simulink model "r2_2f_4x_4a_4k_r366"  (R2012b)
(part 3 of 103)

      | elseif strcmp(mode, 'fields of arbitrary size')
      |     current_names = textscan(strtrim(strrep(strrep(get_param(blk, 'names'), ']', ''), '[', '')), '%s');
      |     current_names = current_names{1};
      |     numios = length(current_names);
      |     if length(current_widths) ~= numios,
      |         error('%d field names specified, but %d widths?', numios, length(current_widths));
      |     end
      | end
      | total_width = 0;
      | for ctr = 1 : length(current_widths),
      |     total_width = total_width + current_widths(ctr);
      | end
      | if total_width > 32,
      |     error('Total width must be 32 or less, set to %d.', total_width);
      | end
      mask Callback arith_types:
      | blk = gcb;
      | mode = get_param(blk, 'mode');
      | current_types = eval(get_param(blk, 'arith_types'));
      | numios = length(current_types);
      | if (strcmp(mode, 'one value') || strcmp(mode, 'fields of equal size')) && (length(current_types) > 1),
      |     error('Only one type may be specified for this mode.');
      | elseif strcmp(mode, 'fields of arbitrary size')
      |     current_names = textscan(strtrim(strrep(strrep(get_param(blk, 'names'), ']', ''), '[', '')), '%s');
      |     current_names = current_names{1};
      |     numios = length(current_names);
      |     if length(current_types) ~= numios,
      |         error('%d field names specified, but %d types?', numios, length(current_types));
      |     end
      | end
      | problem = 0;
      | for ctr = 1 : numios,
      |     t = current_types(ctr);
      |     if (t < 0) || (t > 2),
      |         problem = t;
      |         ctr = numios + 1;
      |     end
      | end
      | if problem ~= 0,
      |     error('Type cannot be %i, must be 0, 1 or 2.', problem);
      | end
      mask Callback bin_pts:
      | blk = gcb;
      | mode = get_param(blk, 'mode');
      | current_bins = eval(get_param(blk, 'bin_pts'));
      | if (strcmp(mode, 'one value') || strcmp(mode, 'fields of equal size')) && (length(current_bins) > 1),
      |     error('Only one binary pt may be specified for this mode.');
      | elseif strcmp(mode, 'fields of arbitrary size')
      |     current_names = textscan(strtrim(strrep(strrep(get_param(blk, 'names'), ']', ''), '[', '')), '%s');
      |     current_names = current_names{1};
      |     numios = length(current_names);
      |     if length(current_bins) ~= numios,
      |         error('%d field names specified, but %d binary pts?', numios, length(current_bins));
      |     end
      | end
  vacc_ld_status0 : Subsystem  Tag=xps:sw_reg  AncestorBlock=xps_library/software register  mask(swreg){mode=one value, io_dir=To Processor, io_delay=1, sample_period=1, names=reg, bitwidths=32, arith_types=0, bin_pts=0, sim_port=off, show_format=off}
      mask prompts: io_dir "I/O direction"; io_delay "I/O delay"; sample_period "Sample period"; names "Name:"; bitwidths "Bitwidth:"; arith_types "Type (ufix=0, fix=1, bool=2):"; bin_pts "Binary pt:"; sim_port "Provide sim input/output?"; show_format "Print format string?"
      mask init:
      | swreg_init(gcb)
      settings: AttributesFormatString=1output
      mask TypeOptions mode: one value | fields of equal size | fields of arbitrary size
      mask Callback mode: swreg_cb(gcb);
      mask TypeOptions io_dir: To Processor | From Processor
      mask Callback io_dir:
      | mask_enables = get_param(gcb, 'MaskEnables');
      | mask_names = get_param(gcb, 'MaskNames');
      | if strcmp(get_param(gcb, 'io_dir'), 'To Processor'),
      |     mask_enables{ismember(mask_names, 'sample_period')} = 'off';
      | else
      |     mask_enables{ismember(mask_names, 'sample_period')} = 'on';
      | end
      | set_param(gcb, 'MaskEnables', mask_enables);
      mask Callback bitwidths:
      | blk = gcb;
      | mode = get_param(blk, 'mode');
      | current_widths = eval(get_param(blk, 'bitwidths'));
      | if (strcmp(mode, 'one value') || strcmp(mode, 'fields of equal size')) && (length(current_widths) > 1),
      |     error('Only one width may be specified for this mode.');
      | elseif strcmp(mode, 'fields of arbitrary size')
      |     current_names = textscan(strtrim(strrep(strrep(get_param(blk, 'names'), ']', ''), '[', '')), '%s');
      |     current_names = current_names{1};
      |     numios = length(current_names);
      |     if length(current_widths) ~= numios,
      |         error('%d field names specified, but %d widths?', numios, length(current_widths));
      |     end
      | end
      | total_width = 0;
      | for ctr = 1 : length(current_widths),
      |     total_width = total_width + current_widths(ctr);
      | end
      | if total_width > 32,
      |     error('Total width must be 32 or less, set to %d.', total_width);
      | end
      mask Callback arith_types:
      | blk = gcb;
      | mode = get_param(blk, 'mode');
      | current_types = eval(get_param(blk, 'arith_types'));
      | numios = length(current_types);
      | if (strcmp(mode, 'one value') || strcmp(mode, 'fields of equal size')) && (length(current_types) > 1),
      |     error('Only one type may be specified for this mode.');
      | elseif strcmp(mode, 'fields of arbitrary size')
      |     current_names = textscan(strtrim(strrep(strrep(get_param(blk, 'names'), ']', ''), '[', '')), '%s');
      |     current_names = current_names{1};
      |     numios = length(current_names);
      |     if length(current_types) ~= numios,
      |         error('%d field names specified, but %d types?', numios, length(current_types));
      |     end
      | end
      | problem = 0;
      | for ctr = 1 : numios,
      |     t = current_types(ctr);
      |     if (t < 0) || (t > 2),
      |         problem = t;
      |         ctr = numios + 1;
      |     end
      | end
      | if problem ~= 0,
      |     error('Type cannot be %i, must be 0, 1 or 2.', problem);
      | end
      mask Callback bin_pts:
      | blk = gcb;
      | mode = get_param(blk, 'mode');
      | current_bins = eval(get_param(blk, 'bin_pts'));
      | if (strcmp(mode, 'one value') || strcmp(mode, 'fields of equal size')) && (length(current_bins) > 1),
      |     error('Only one binary pt may be specified for this mode.');
      | elseif strcmp(mode, 'fields of arbitrary size')
      |     current_names = textscan(strtrim(strrep(strrep(get_param(blk, 'names'), ']', ''), '[', '')), '%s');
      |     current_names = current_names{1};
      |     numios = length(current_names);
      |     if length(current_bins) ~= numios,
      |         error('%d field names specified, but %d binary pts?', numios, length(current_bins));
      |     end
      | end
  vacc_ld_status1 : Subsystem  Tag=xps:sw_reg  AncestorBlock=xps_library/software register  mask(swreg){mode=one value, io_dir=To Processor, io_delay=1, sample_period=1, names=reg, bitwidths=32, arith_types=0, bin_pts=0, sim_port=off, show_format=off}
      mask prompts: io_dir "I/O direction"; io_delay "I/O delay"; sample_period "Sample period"; names "Name:"; bitwidths "Bitwidth:"; arith_types "Type (ufix=0, fix=1, bool=2):"; bin_pts "Binary pt:"; sim_port "Provide sim input/output?"; show_format "Print format string?"
      mask init:
      | swreg_init(gcb)
      settings: AttributesFormatString=1output
      mask TypeOptions mode: one value | fields of equal size | fields of arbitrary size
      mask Callback mode: swreg_cb(gcb);
      mask TypeOptions io_dir: To Processor | From Processor
      mask Callback io_dir:
      | mask_enables = get_param(gcb, 'MaskEnables');
      | mask_names = get_param(gcb, 'MaskNames');
      | if strcmp(get_param(gcb, 'io_dir'), 'To Processor'),
      |     mask_enables{ismember(mask_names, 'sample_period')} = 'off';
      | else
      |     mask_enables{ismember(mask_names, 'sample_period')} = 'on';
      | end
      | set_param(gcb, 'MaskEnables', mask_enables);
      mask Callback bitwidths:
      | blk = gcb;
      | mode = get_param(blk, 'mode');
      | current_widths = eval(get_param(blk, 'bitwidths'));
      | if (strcmp(mode, 'one value') || strcmp(mode, 'fields of equal size')) && (length(current_widths) > 1),
      |     error('Only one width may be specified for this mode.');
      | elseif strcmp(mode, 'fields of arbitrary size')
      |     current_names = textscan(strtrim(strrep(strrep(get_param(blk, 'names'), ']', ''), '[', '')), '%s');
      |     current_names = current_names{1};
      |     numios = length(current_names);
      |     if length(current_widths) ~= numios,
      |         error('%d field names specified, but %d widths?', numios, length(current_widths));
      |     end
      | end
      | total_width = 0;
      | for ctr = 1 : length(current_widths),
      |     total_width = total_width + current_widths(ctr);
      | end
      | if total_width > 32,
      |     error('Total width must be 32 or less, set to %d.', total_width);
      | end
      mask Callback arith_types:
      | blk = gcb;
      | mode = get_param(blk, 'mode');
      | current_types = eval(get_param(blk, 'arith_types'));
      | numios = length(current_types);
      | if (strcmp(mode, 'one value') || strcmp(mode, 'fields of equal size')) && (length(current_types) > 1),
      |     error('Only one type may be specified for this mode.');
      | elseif strcmp(mode, 'fields of arbitrary size')
      |     current_names = textscan(strtrim(strrep(strrep(get_param(blk, 'names'), ']', ''), '[', '')), '%s');
      |     current_names = current_names{1};
      |     numios = length(current_names);
      |     if length(current_types) ~= numios,
      |         error('%d field names specified, but %d types?', numios, length(current_types));
      |     end
      | end
      | problem = 0;
      | for ctr = 1 : numios,
      |     t = current_types(ctr);
      |     if (t < 0) || (t > 2),
      |         problem = t;
      |         ctr = numios + 1;
      |     end
      | end
      | if problem ~= 0,
      |     error('Type cannot be %i, must be 0, 1 or 2.', problem);
      | end
      mask Callback bin_pts:
      | blk = gcb;
      | mode = get_param(blk, 'mode');
      | current_bins = eval(get_param(blk, 'bin_pts'));
      | if (strcmp(mode, 'one value') || strcmp(mode, 'fields of equal size')) && (length(current_bins) > 1),
      |     error('Only one binary pt may be specified for this mode.');
      | elseif strcmp(mode, 'fields of arbitrary size')
      |     current_names = textscan(strtrim(strrep(strrep(get_param(blk, 'names'), ']', ''), '[', '')), '%s');
      |     current_names = current_names{1};
      |     numios = length(current_names);
      |     if length(current_bins) ~= numios,
      |         error('%d field names specified, but %d binary pts?', numios, length(current_bins));
      |     end
      | end
  vacc_ld_status2 : Subsystem  Tag=xps:sw_reg  AncestorBlock=xps_library/software register  mask(swreg){mode=one value, io_dir=To Processor, io_delay=1, sample_period=1, names=reg, bitwidths=32, arith_types=0, bin_pts=0, sim_port=off, show_format=off}
      mask prompts: io_dir "I/O direction"; io_delay "I/O delay"; sample_period "Sample period"; names "Name:"; bitwidths "Bitwidth:"; arith_types "Type (ufix=0, fix=1, bool=2):"; bin_pts "Binary pt:"; sim_port "Provide sim input/output?"; show_format "Print format string?"
      mask init:
      | swreg_init(gcb)
      settings: AttributesFormatString=1output
      mask TypeOptions mode: one value | fields of equal size | fields of arbitrary size
      mask Callback mode: swreg_cb(gcb);
      mask TypeOptions io_dir: To Processor | From Processor
      mask Callback io_dir:
      | mask_enables = get_param(gcb, 'MaskEnables');
      | mask_names = get_param(gcb, 'MaskNames');
      | if strcmp(get_param(gcb, 'io_dir'), 'To Processor'),
      |     mask_enables{ismember(mask_names, 'sample_period')} = 'off';
      | else
      |     mask_enables{ismember(mask_names, 'sample_period')} = 'on';
      | end
      | set_param(gcb, 'MaskEnables', mask_enables);
      mask Callback bitwidths:
      | blk = gcb;
      | mode = get_param(blk, 'mode');
      | current_widths = eval(get_param(blk, 'bitwidths'));
      | if (strcmp(mode, 'one value') || strcmp(mode, 'fields of equal size')) && (length(current_widths) > 1),
      |     error('Only one width may be specified for this mode.');
      | elseif strcmp(mode, 'fields of arbitrary size')
      |     current_names = textscan(strtrim(strrep(strrep(get_param(blk, 'names'), ']', ''), '[', '')), '%s');
      |     current_names = current_names{1};
      |     numios = length(current_names);
      |     if length(current_widths) ~= numios,
      |         error('%d field names specified, but %d widths?', numios, length(current_widths));
      |     end
      | end
      | total_width = 0;
      | for ctr = 1 : length(current_widths),
      |     total_width = total_width + current_widths(ctr);
      | end
      | if total_width > 32,
      |     error('Total width must be 32 or less, set to %d.', total_width);
      | end
      mask Callback arith_types:
      | blk = gcb;
      | mode = get_param(blk, 'mode');
      | current_types = eval(get_param(blk, 'arith_types'));
      | numios = length(current_types);
      | if (strcmp(mode, 'one value') || strcmp(mode, 'fields of equal size')) && (length(current_types) > 1),
      |     error('Only one type may be specified for this mode.');
      | elseif strcmp(mode, 'fields of arbitrary size')
      |     current_names = textscan(strtrim(strrep(strrep(get_param(blk, 'names'), ']', ''), '[', '')), '%s');
      |     current_names = current_names{1};
      |     numios = length(current_names);
      |     if length(current_types) ~= numios,
      |         error('%d field names specified, but %d types?', numios, length(current_types));
      |     end
      | end
      | problem = 0;
      | for ctr = 1 : numios,
      |     t = current_types(ctr);
      |     if (t < 0) || (t > 2),
      |         problem = t;
      |         ctr = numios + 1;
      |     end
      | end
      | if problem ~= 0,
      |     error('Type cannot be %i, must be 0, 1 or 2.', problem);
      | end
      mask Callback bin_pts:
      | blk = gcb;
      | mode = get_param(blk, 'mode');
      | current_bins = eval(get_param(blk, 'bin_pts'));
      | if (strcmp(mode, 'one value') || strcmp(mode, 'fields of equal size')) && (length(current_bins) > 1),
      |     error('Only one binary pt may be specified for this mode.');
      | elseif strcmp(mode, 'fields of arbitrary size')
      |     current_names = textscan(strtrim(strrep(strrep(get_param(blk, 'names'), ']', ''), '[', '')), '%s');
      |     current_names = current_names{1};
      |     numios = length(current_names);
      |     if length(current_bins) ~= numios,
      |         error('%d field names specified, but %d binary pts?', numios, length(current_bins));
      |     end
      | end
  vacc_ld_status3 : Subsystem  Tag=xps:sw_reg  AncestorBlock=xps_library/software register  mask(swreg){mode=one value, io_dir=To Processor, io_delay=1, sample_period=1, names=reg, bitwidths=32, arith_types=0, bin_pts=0, sim_port=off, show_format=off}
      mask prompts: io_dir "I/O direction"; io_delay "I/O delay"; sample_period "Sample period"; names "Name:"; bitwidths "Bitwidth:"; arith_types "Type (ufix=0, fix=1, bool=2):"; bin_pts "Binary pt:"; sim_port "Provide sim input/output?"; show_format "Print format string?"
      mask init:
      | swreg_init(gcb)
      settings: AttributesFormatString=1output
      mask TypeOptions mode: one value | fields of equal size | fields of arbitrary size
      mask Callback mode: swreg_cb(gcb);
      mask TypeOptions io_dir: To Processor | From Processor
      mask Callback io_dir:
      | mask_enables = get_param(gcb, 'MaskEnables');
      | mask_names = get_param(gcb, 'MaskNames');
      | if strcmp(get_param(gcb, 'io_dir'), 'To Processor'),
      |     mask_enables{ismember(mask_names, 'sample_period')} = 'off';
      | else
      |     mask_enables{ismember(mask_names, 'sample_period')} = 'on';
      | end
      | set_param(gcb, 'MaskEnables', mask_enables);
      mask Callback bitwidths:
      | blk = gcb;
      | mode = get_param(blk, 'mode');
      | current_widths = eval(get_param(blk, 'bitwidths'));
      | if (strcmp(mode, 'one value') || strcmp(mode, 'fields of equal size')) && (length(current_widths) > 1),
      |     error('Only one width may be specified for this mode.');
      | elseif strcmp(mode, 'fields of arbitrary size')
      |     current_names = textscan(strtrim(strrep(strrep(get_param(blk, 'names'), ']', ''), '[', '')), '%s');
      |     current_names = current_names{1};
      |     numios = length(current_names);
      |     if length(current_widths) ~= numios,
      |         error('%d field names specified, but %d widths?', numios, length(current_widths));
      |     end
      | end
      | total_width = 0;
      | for ctr = 1 : length(current_widths),
      |     total_width = total_width + current_widths(ctr);
      | end
      | if total_width > 32,
      |     error('Total width must be 32 or less, set to %d.', total_width);
      | end
      mask Callback arith_types:
      | blk = gcb;
      | mode = get_param(blk, 'mode');
      | current_types = eval(get_param(blk, 'arith_types'));
      | numios = length(current_types);
      | if (strcmp(mode, 'one value') || strcmp(mode, 'fields of equal size')) && (length(current_types) > 1),
      |     error('Only one type may be specified for this mode.');
      | elseif strcmp(mode, 'fields of arbitrary size')
      |     current_names = textscan(strtrim(strrep(strrep(get_param(blk, 'names'), ']', ''), '[', '')), '%s');
      |     current_names = current_names{1};
      |     numios = length(current_names);
      |     if length(current_types) ~= numios,
      |         error('%d field names specified, but %d types?', numios, length(current_types));
      |     end
      | end
      | problem = 0;
      | for ctr = 1 : numios,
      |     t = current_types(ctr);
      |     if (t < 0) || (t > 2),
      |         problem = t;
      |         ctr = numios + 1;
      |     end
      | end
      | if problem ~= 0,
      |     error('Type cannot be %i, must be 0, 1 or 2.', problem);
      | end
      mask Callback bin_pts:
      | blk = gcb;
      | mode = get_param(blk, 'mode');
      | current_bins = eval(get_param(blk, 'bin_pts'));
      | if (strcmp(mode, 'one value') || strcmp(mode, 'fields of equal size')) && (length(current_bins) > 1),
      |     error('Only one binary pt may be specified for this mode.');
      | elseif strcmp(mode, 'fields of arbitrary size')
      |     current_names = textscan(strtrim(strrep(strrep(get_param(blk, 'names'), ']', ''), '[', '')), '%s');
      |     current_names = current_names{1};
      |     numios = length(current_names);
      |     if length(current_bins) ~= numios,
      |         error('%d field names specified, but %d binary pts?', numios, length(current_bins));
      |     end
      | end
  vacc_monitor : Subsystem
  vacc_monitor1 : Subsystem
  vacc_monitor2 : Subsystem
  vacc_monitor3 : Subsystem
  vacc_monitor4 : Subsystem
  vacc_monitor5 : Subsystem
  vacc_monitor6 : Subsystem
  vacc_monitor7 : Subsystem
  vacc_time_lsw : Subsystem  Tag=xps:sw_reg  AncestorBlock=xps_library/software register  mask(swreg){mode=one value, io_dir=From Processor, io_delay=1, sample_period=1, names=reg, bitwidths=32, arith_types=0, bin_pts=0, sim_port=on, show_format=off}
      mask prompts: io_dir "I/O direction"; io_delay "I/O delay"; sample_period "Sample period"; names "Name:"; bitwidths "Bitwidth:"; arith_types "Type (ufix=0, fix=1, bool=2):"; bin_pts "Binary pt:"; sim_port "Provide sim input/output?"; show_format "Print format string?"
      mask init:
      | swreg_init(gcb)
      settings: AttributesFormatString=1input
      mask TypeOptions mode: one value | fields of equal size | fields of arbitrary size
      mask Callback mode: swreg_cb(gcb);
      mask TypeOptions io_dir: To Processor | From Processor
      mask Callback io_dir:
      | mask_enables = get_param(gcb, 'MaskEnables');
      | mask_names = get_param(gcb, 'MaskNames');
      | if strcmp(get_param(gcb, 'io_dir'), 'To Processor'),
      |     mask_enables{ismember(mask_names, 'sample_period')} = 'off';
      | else
      |     mask_enables{ismember(mask_names, 'sample_period')} = 'on';
      | end
      | set_param(gcb, 'MaskEnables', mask_enables);
      mask Callback bitwidths:
      | blk = gcb;
      | mode = get_param(blk, 'mode');
      | current_widths = eval(get_param(blk, 'bitwidths'));
      | if (strcmp(mode, 'one value') || strcmp(mode, 'fields of equal size')) && (length(current_widths) > 1),
      |     error('Only one width may be specified for this mode.');
      | elseif strcmp(mode, 'fields of arbitrary size')
      |     current_names = textscan(strtrim(strrep(strrep(get_param(blk, 'names'), ']', ''), '[', '')), '%s');
      |     current_names = current_names{1};
      |     numios = length(current_names);
      |     if length(current_widths) ~= numios,
      |         error('%d field names specified, but %d widths?', numios, length(current_widths));
      |     end
      | end
      | total_width = 0;
      | for ctr = 1 : length(current_widths),
      |     total_width = total_width + current_widths(ctr);
      | end
      | if total_width > 32,
      |     error('Total width must be 32 or less, set to %d.', total_width);
      | end
      mask Callback arith_types:
      | blk = gcb;
      | mode = get_param(blk, 'mode');
      | current_types = eval(get_param(blk, 'arith_types'));
      | numios = length(current_types);
      | if (strcmp(mode, 'one value') || strcmp(mode, 'fields of equal size')) && (length(current_types) > 1),
      |     error('Only one type may be specified for this mode.');
      | elseif strcmp(mode, 'fields of arbitrary size')
      |     current_names = textscan(strtrim(strrep(strrep(get_param(blk, 'names'), ']', ''), '[', '')), '%s');
      |     current_names = current_names{1};
      |     numios = length(current_names);
      |     if length(current_types) ~= numios,
      |         error('%d field names specified, but %d types?', numios, length(current_types));
      |     end
      | end
      | problem = 0;
      | for ctr = 1 : numios,
      |     t = current_types(ctr);
      |     if (t < 0) || (t > 2),
      |         problem = t;
      |         ctr = numios + 1;
      |     end
      | end
      | if problem ~= 0,
      |     error('Type cannot be %i, must be 0, 1 or 2.', problem);
      | end
      mask Callback bin_pts:
      | blk = gcb;
      | mode = get_param(blk, 'mode');
      | current_bins = eval(get_param(blk, 'bin_pts'));
      | if (strcmp(mode, 'one value') || strcmp(mode, 'fields of equal size')) && (length(current_bins) > 1),
      |     error('Only one binary pt may be specified for this mode.');
      | elseif strcmp(mode, 'fields of arbitrary size')
      |     current_names = textscan(strtrim(strrep(strrep(get_param(blk, 'names'), ']', ''), '[', '')), '%s');
      |     current_names = current_names{1};
      |     numios = length(current_names);
      |     if length(current_bins) ~= numios,
      |         error('%d field names specified, but %d binary pts?', numios, length(current_bins));
      |     end
      | end
  vacc_time_msw : Subsystem  Tag=xps:sw_reg  AncestorBlock=xps_library/software register  mask(swreg){mode=fields of arbitrary size, io_dir=From Processor, io_delay=1, sample_period=1, names=[arm msw], bitwidths=[1 16], arith_types=[2 0], bin_pts=[0 0], sim_port=off, show_format=off}
      mask prompts: io_dir "I/O direction"; io_delay "I/O delay"; sample_period "Sample period"; names "Names [msb ... lsb]:"; bitwidths "Bitwidths [msb ... lsb]:"; arith_types "Types (ufix=0, fix=1, bool=2) [msb ... lsb]:"; bin_pts "Binary pts [msb ... lsb]:"; sim_port "Provide sim input/output?"; show_format "Print format string?"
      mask init:
      | swreg_init(gcb)
      settings: AttributesFormatString=2 inputs
      mask TypeOptions mode: one value | fields of equal size | fields of arbitrary size
      mask Callback mode: swreg_cb(gcb);
      mask TypeOptions io_dir: To Processor | From Processor
      mask Callback io_dir:
      | mask_enables = get_param(gcb, 'MaskEnables');
      | mask_names = get_param(gcb, 'MaskNames');
      | if strcmp(get_param(gcb, 'io_dir'), 'To Processor'),
      |     mask_enables{ismember(mask_names, 'sample_period')} = 'off';
      | else
      |     mask_enables{ismember(mask_names, 'sample_period')} = 'on';
      | end
      | set_param(gcb, 'MaskEnables', mask_enables);
      mask Callback bitwidths:
      | blk = gcb;
      | mode = get_param(blk, 'mode');
      | current_widths = eval(get_param(blk, 'bitwidths'));
      | if (strcmp(mode, 'one value') || strcmp(mode, 'fields of equal size')) && (length(current_widths) > 1),
      |     error('Only one width may be specified for this mode.');
      | elseif strcmp(mode, 'fields of arbitrary size')
      |     current_names = textscan(strtrim(strrep(strrep(get_param(blk, 'names'), ']', ''), '[', '')), '%s');
      |     current_names = current_names{1};
      |     numios = length(current_names);
      |     if length(current_widths) ~= numios,
      |         error('%d field names specified, but %d widths?', numios, length(current_widths));
      |     end
      | end
      | total_width = 0;
      | for ctr = 1 : length(current_widths),
      |     total_width = total_width + current_widths(ctr);
      | end
      | if total_width > 32,
      |     error('Total width must be 32 or less, set to %d.', total_width);
      | end
      mask Callback arith_types:
      | blk = gcb;
      | mode = get_param(blk, 'mode');
      | current_types = eval(get_param(blk, 'arith_types'));
      | numios = length(current_types);
      | if (strcmp(mode, 'one value') || strcmp(mode, 'fields of equal size')) && (length(current_types) > 1),
      |     error('Only one type may be specified for this mode.');
      | elseif strcmp(mode, 'fields of arbitrary size')
      |     current_names = textscan(strtrim(strrep(strrep(get_param(blk, 'names'), ']', ''), '[', '')), '%s');
      |     current_names = current_names{1};
      |     numios = length(current_names);
      |     if length(current_types) ~= numios,
      |         error('%d field names specified, but %d types?', numios, length(current_types));
      |     end
      | end
      | problem = 0;
      | for ctr = 1 : numios,
      |     t = current_types(ctr);
      |     if (t < 0) || (t > 2),
      |         problem = t;
      |         ctr = numios + 1;
      |     end
      | end
      | if problem ~= 0,
      |     error('Type cannot be %i, must be 0, 1 or 2.', problem);
      | end
      mask Callback bin_pts:
      | blk = gcb;
      | mode = get_param(blk, 'mode');
      | current_bins = eval(get_param(blk, 'bin_pts'));
      | if (strcmp(mode, 'one value') || strcmp(mode, 'fields of equal size')) && (length(current_bins) > 1),
      |     error('Only one binary pt may be specified for this mode.');
      | elseif strcmp(mode, 'fields of arbitrary size')
      |     current_names = textscan(strtrim(strrep(strrep(get_param(blk, 'names'), ']', ''), '[', '')), '%s');
      |     current_names = current_names{1};
      |     numios = length(current_names);
      |     if length(current_bins) ~= numios,
      |         error('%d field names specified, but %d binary pts?', numios, length(current_bins));
      |     end
      | end
  vacc_tvg0 : Subsystem  AncestorBlock=casper_library/Accumulators/vacc_tvg  mask{len=(4*(4+1))/2*8*2^(12-4)}
      mask prompts: len "Number of Vectors"
      mask init:
      | fmtstr = sprintf('Vector Length: %d', len);
      | set_param(gcb, 'AttributesFormatString', fmtstr);
      settings: AttributesFormatString=Vector Length: 20480
  vacc_tvg1 : Subsystem  AncestorBlock=casper_library/Accumulators/vacc_tvg  mask{len=(4*(4+1))/2*8*2^(12-4)}
      mask prompts: len "Number of Vectors"
      mask init:
      | fmtstr = sprintf('Vector Length: %d', len);
      | set_param(gcb, 'AttributesFormatString', fmtstr);
      settings: AttributesFormatString=Vector Length: 20480
  vacc_tvg2 : Subsystem  AncestorBlock=casper_library/Accumulators/vacc_tvg  mask{len=(4*(4+1))/2*8*2^(12-4)}
      mask prompts: len "Number of Vectors"
      mask init:
      | fmtstr = sprintf('Vector Length: %d', len);
      | set_param(gcb, 'AttributesFormatString', fmtstr);
      settings: AttributesFormatString=Vector Length: 20480
  vacc_tvg3 : Subsystem  AncestorBlock=casper_library/Accumulators/vacc_tvg  mask{len=(4*(4+1))/2*8*2^(12-4)}
      mask prompts: len "Number of Vectors"
      mask init:
      | fmtstr = sprintf('Vector Length: %d', len);
      | set_param(gcb, 'AttributesFormatString', fmtstr);
      settings: AttributesFormatString=Vector Length: 20480
  xeng0 : Subsystem  Tag=casper:xeng  AncestorBlock=casper_library_correlator/xeng  mask(xeng){n_ants=4, n_bits=8, acc_len=256, demux_factor=8, add_latency=2, mult_latency=4, bram_latency=6, use_ded_mult=1, use_bram_delay=1}
      mask prompts: n_ants "Number of antennas"; n_bits "Bit-width of samples in"; acc_len "Accumulation length"; add_latency "Adder latency"; mult_latency "Multiplier latency"; bram_latency "BRAM latency"; use_ded_mult "Implementation: Multiplier type (0=slices 1=embedded 2=bram)"; use_bram_delay "Implementation: Delay type (0=SLR, 1=BRAM)"
      mask help: CASPER X engine with added internal valid data masking functionality, descramble and integral demux. Based on Aaron Parsons' and Lynn Urry's original X engine design.
      mask init:
      | xeng_init(gcb, ...
      |     'n_ants', n_ants, ...
      |     'n_bits', n_bits, ...
      |     'acc_len', acc_len, ...
      |     'demux_factor', demux_factor, ...
      |     'add_latency', add_latency, ...
      |     'mult_latency', mult_latency, ...
      |     'bram_latency', bram_latency, ...
      |     'use_ded_mult', use_ded_mult, ...
      |     'use_bram_delay', use_bram_delay);
      settings: AttributesFormatString=n_ant=4, bits=8, mult_typ=1, bram_typ=1
      mask TypeOptions demux_factor: 1 | 2 | 4 | 8
  xeng1 : Subsystem  Tag=casper:xeng  AncestorBlock=casper_library_correlator/xeng  mask(xeng){n_ants=4, n_bits=8, acc_len=256, demux_factor=8, add_latency=2, mult_latency=4, bram_latency=6, use_ded_mult=1, use_bram_delay=1}
      mask prompts: n_ants "Number of antennas"; n_bits "Bit-width of samples in"; acc_len "Accumulation length"; add_latency "Adder latency"; mult_latency "Multiplier latency"; bram_latency "BRAM latency"; use_ded_mult "Implementation: Multiplier type (0=slices 1=embedded 2=bram)"; use_bram_delay "Implementation: Delay type (0=SLR, 1=BRAM)"
      mask help: CASPER X engine with added internal valid data masking functionality, descramble and integral demux. Based on Aaron Parsons' and Lynn Urry's original X engine design.
      mask init: same as r2_2f_4x_4a_4k_r366/xeng0
      settings: AttributesFormatString=n_ant=4, bits=8, mult_typ=1, bram_typ=1
      mask TypeOptions demux_factor: 1 | 2 | 4 | 8
  xeng2 : Subsystem  Tag=casper:xeng  AncestorBlock=casper_library_correlator/xeng  mask(xeng){n_ants=4, n_bits=8, acc_len=256, demux_factor=8, add_latency=2, mult_latency=4, bram_latency=6, use_ded_mult=1, use_bram_delay=1}
      mask prompts: n_ants "Number of antennas"; n_bits "Bit-width of samples in"; acc_len "Accumulation length"; add_latency "Adder latency"; mult_latency "Multiplier latency"; bram_latency "BRAM latency"; use_ded_mult "Implementation: Multiplier type (0=slices 1=embedded 2=bram)"; use_bram_delay "Implementation: Delay type (0=SLR, 1=BRAM)"
      mask help: CASPER X engine with added internal valid data masking functionality, descramble and integral demux. Based on Aaron Parsons' and Lynn Urry's original X engine design.
      mask init: same as r2_2f_4x_4a_4k_r366/xeng0
      settings: AttributesFormatString=n_ant=4, bits=8, mult_typ=1, bram_typ=1
      mask TypeOptions demux_factor: 1 | 2 | 4 | 8
  xeng3 : Subsystem  Tag=casper:xeng  AncestorBlock=casper_library_correlator/xeng  mask(xeng){n_ants=4, n_bits=8, acc_len=256, demux_factor=8, add_latency=2, mult_latency=4, bram_latency=6, use_ded_mult=1, use_bram_delay=1}
      mask prompts: n_ants "Number of antennas"; n_bits "Bit-width of samples in"; acc_len "Accumulation length"; add_latency "Adder latency"; mult_latency "Multiplier latency"; bram_latency "BRAM latency"; use_ded_mult "Implementation: Multiplier type (0=slices 1=embedded 2=bram)"; use_bram_delay "Implementation: Delay type (0=SLR, 1=BRAM)"
      mask help: CASPER X engine with added internal valid data masking functionality, descramble and integral demux. Based on Aaron Parsons' and Lynn Urry's original X engine design.
      mask init: same as r2_2f_4x_4a_4k_r366/xeng0
      settings: AttributesFormatString=n_ant=4, bits=8, mult_typ=1, bram_typ=1
      mask TypeOptions demux_factor: 1 | 2 | 4 | 8
  xeng_tvg0 : Subsystem  AncestorBlock=casper_library/Correlator/xeng_tvg  mask{ant_bits=2, x_int_bits=8, sync_period=16}
      mask prompts: ant_bits "Number of Antennas (2^?):"; x_int_bits "X Integration Length (2^?):"; sync_period "Sync Pulse Period (2^?):"
  xeng_tvg1 : Subsystem  AncestorBlock=casper_library/Correlator/xeng_tvg  mask{ant_bits=2, x_int_bits=8, sync_period=16}
      mask prompts: ant_bits "Number of Antennas (2^?):"; x_int_bits "X Integration Length (2^?):"; sync_period "Sync Pulse Period (2^?):"
  xeng_tvg2 : Subsystem  AncestorBlock=casper_library/Correlator/xeng_tvg  mask{ant_bits=2, x_int_bits=8, sync_period=16}
      mask prompts: ant_bits "Number of Antennas (2^?):"; x_int_bits "X Integration Length (2^?):"; sync_period "Sync Pulse Period (2^?):"
  xeng_tvg3 : Subsystem  AncestorBlock=casper_library/Correlator/xeng_tvg  mask{ant_bits=2, x_int_bits=8, sync_period=16}
      mask prompts: ant_bits "Number of Antennas (2^?):"; x_int_bits "X Integration Length (2^?):"; sync_period "Sync Pulse Period (2^?):"
  xstatus0 : Subsystem  Tag=xps:sw_reg  AncestorBlock=xps_library/software register  mask(swreg){mode=fields of equal size, io_dir=To Processor, io_delay=1, sample_period=1, names=[gbe_down rx_dest_err feng_rx_err fft_err feng_qdr_err feng_chk_err adc_over noise_diode_en vacc_err rx_bad_pkt rx_bad_frame tx_over xeng_bad_dat pack_err], bitwidths=1, arith_types=2, bin_pts=0, sim_port=off, show_format=off}
      mask prompts: io_dir "I/O direction"; io_delay "I/O delay"; sample_period "Sample period"; names "Names [msb ... lsb]:"; bitwidths "Bitwidth:"; arith_types "Type (ufix=0, fix=1, bool=2):"; bin_pts "Binary pt:"; sim_port "Provide sim input/output?"; show_format "Print format string?"
      mask init:
      | swreg_init(gcb)
      settings: AttributesFormatString=14 outputs
      mask TypeOptions mode: one value | fields of equal size | fields of arbitrary size
      mask Callback mode: swreg_cb(gcb);
      mask TypeOptions io_dir: To Processor | From Processor
      mask Callback io_dir:
      | mask_enables = get_param(gcb, 'MaskEnables');
      | mask_names = get_param(gcb, 'MaskNames');
      | if strcmp(get_param(gcb, 'io_dir'), 'To Processor'),
      |     mask_enables{ismember(mask_names, 'sample_period')} = 'off';
      | else
      |     mask_enables{ismember(mask_names, 'sample_period')} = 'on';
      | end
      | set_param(gcb, 'MaskEnables', mask_enables);
      mask Callback bitwidths:
      | blk = gcb;
      | mode = get_param(blk, 'mode');
      | current_widths = eval(get_param(blk, 'bitwidths'));
      | if (strcmp(mode, 'one value') || strcmp(mode, 'fields of equal size')) && (length(current_widths) > 1),
      |     error('Only one width may be specified for this mode.');
      | elseif strcmp(mode, 'fields of arbitrary size')
      |     current_names = textscan(strtrim(strrep(strrep(get_param(blk, 'names'), ']', ''), '[', '')), '%s');
      |     current_names = current_names{1};
      |     numios = length(current_names);
      |     if length(current_widths) ~= numios,
      |         error('%d field names specified, but %d widths?', numios, length(current_widths));
      |     end
      | end
      | total_width = 0;
      | for ctr = 1 : length(current_widths),
      |     total_width = total_width + current_widths(ctr);
      | end
      | if total_width > 32,
      |     error('Total width must be 32 or less, set to %d.', total_width);
      | end
      mask Callback arith_types:
      | blk = gcb;
      | mode = get_param(blk, 'mode');
      | current_types = eval(get_param(blk, 'arith_types'));
      | numios = length(current_types);
      | if (strcmp(mode, 'one value') || strcmp(mode, 'fields of equal size')) && (length(current_types) > 1),
      |     error('Only one type may be specified for this mode.');
      | elseif strcmp(mode, 'fields of arbitrary size')
      |     current_names = textscan(strtrim(strrep(strrep(get_param(blk, 'names'), ']', ''), '[', '')), '%s');
      |     current_names = current_names{1};
      |     numios = length(current_names);
      |     if length(current_types) ~= numios,
      |         error('%d field names specified, but %d types?', numios, length(current_types));
      |     end
      | end
      | problem = 0;
      | for ctr = 1 : numios,
      |     t = current_types(ctr);
      |     if (t < 0) || (t > 2),
      |         problem = t;
      |         ctr = numios + 1;
      |     end
      | end
      | if problem ~= 0,
      |     error('Type cannot be %i, must be 0, 1 or 2.', problem);
      | end
      mask Callback bin_pts:
      | blk = gcb;
      | mode = get_param(blk, 'mode');
      | current_bins = eval(get_param(blk, 'bin_pts'));
      | if (strcmp(mode, 'one value') || strcmp(mode, 'fields of equal size')) && (length(current_bins) > 1),
      |     error('Only one binary pt may be specified for this mode.');
      | elseif strcmp(mode, 'fields of arbitrary size')
      |     current_names = textscan(strtrim(strrep(strrep(get_param(blk, 'names'), ']', ''), '[', '')), '%s');
      |     current_names = current_names{1};
      |     numios = length(current_names);
      |     if length(current_bins) ~= numios,
      |         error('%d field names specified, but %d binary pts?', numios, length(current_bins));
      |     end
      | end
  xstatus1 : Subsystem  Tag=xps:sw_reg  AncestorBlock=xps_library/software register  mask(swreg){mode=fields of equal size, io_dir=To Processor, io_delay=1, sample_period=1, names=[gbe_down rx_dest_err feng_rx_err fft_err feng_qdr_err feng_chk_err adc_over noise_diode_en vacc_err rx_bad_pkt rx_bad_frame tx_over xeng_bad_dat pack_err], bitwidths=1, arith_types=2, bin_pts=0, sim_port=off, show_format=off}
      mask prompts: io_dir "I/O direction"; io_delay "I/O delay"; sample_period "Sample period"; names "Names [msb ... lsb]:"; bitwidths "Bitwidth:"; arith_types "Type (ufix=0, fix=1, bool=2):"; bin_pts "Binary pt:"; sim_port "Provide sim input/output?"; show_format "Print format string?"
      mask init:
      | swreg_init(gcb)
      settings: AttributesFormatString=14 outputs
      mask TypeOptions mode: one value | fields of equal size | fields of arbitrary size
      mask Callback mode: swreg_cb(gcb);
      mask TypeOptions io_dir: To Processor | From Processor
      mask Callback io_dir:
      | mask_enables = get_param(gcb, 'MaskEnables');
      | mask_names = get_param(gcb, 'MaskNames');
      | if strcmp(get_param(gcb, 'io_dir'), 'To Processor'),
      |     mask_enables{ismember(mask_names, 'sample_period')} = 'off';
      | else
      |     mask_enables{ismember(mask_names, 'sample_period')} = 'on';
      | end
      | set_param(gcb, 'MaskEnables', mask_enables);
      mask Callback bitwidths:
      | blk = gcb;
      | mode = get_param(blk, 'mode');
      | current_widths = eval(get_param(blk, 'bitwidths'));
      | if (strcmp(mode, 'one value') || strcmp(mode, 'fields of equal size')) && (length(current_widths) > 1),
      |     error('Only one width may be specified for this mode.');
      | elseif strcmp(mode, 'fields of arbitrary size')
      |     current_names = textscan(strtrim(strrep(strrep(get_param(blk, 'names'), ']', ''), '[', '')), '%s');
      |     current_names = current_names{1};
      |     numios = length(current_names);
      |     if length(current_widths) ~= numios,
      |         error('%d field names specified, but %d widths?', numios, length(current_widths));
      |     end
      | end
      | total_width = 0;
      | for ctr = 1 : length(current_widths),
      |     total_width = total_width + current_widths(ctr);
      | end
      | if total_width > 32,
      |     error('Total width must be 32 or less, set to %d.', total_width);
      | end
      mask Callback arith_types:
      | blk = gcb;
      | mode = get_param(blk, 'mode');
      | current_types = eval(get_param(blk, 'arith_types'));
      | numios = length(current_types);
      | if (strcmp(mode, 'one value') || strcmp(mode, 'fields of equal size')) && (length(current_types) > 1),
      |     error('Only one type may be specified for this mode.');
      | elseif strcmp(mode, 'fields of arbitrary size')
      |     current_names = textscan(strtrim(strrep(strrep(get_param(blk, 'names'), ']', ''), '[', '')), '%s');
      |     current_names = current_names{1};
      |     numios = length(current_names);
      |     if length(current_types) ~= numios,
      |         error('%d field names specified, but %d types?', numios, length(current_types));
      |     end
      | end
      | problem = 0;
      | for ctr = 1 : numios,
      |     t = current_types(ctr);
      |     if (t < 0) || (t > 2),
      |         problem = t;
      |         ctr = numios + 1;
      |     end
      | end
      | if problem ~= 0,
      |     error('Type cannot be %i, must be 0, 1 or 2.', problem);
      | end
      mask Callback bin_pts:
      | blk = gcb;
      | mode = get_param(blk, 'mode');
      | current_bins = eval(get_param(blk, 'bin_pts'));
      | if (strcmp(mode, 'one value') || strcmp(mode, 'fields of equal size')) && (length(current_bins) > 1),
      |     error('Only one binary pt may be specified for this mode.');
      | elseif strcmp(mode, 'fields of arbitrary size')
      |     current_names = textscan(strtrim(strrep(strrep(get_param(blk, 'names'), ']', ''), '[', '')), '%s');
      |     current_names = current_names{1};
      |     numios = length(current_names);
      |     if length(current_bins) ~= numios,
      |         error('%d field names specified, but %d binary pts?', numios, length(current_bins));
      |     end
      | end
  xstatus2 : Subsystem  Tag=xps:sw_reg  AncestorBlock=xps_library/software register  mask(swreg){mode=fields of equal size, io_dir=To Processor, io_delay=1, sample_period=1, names=[gbe_down rx_dest_err feng_rx_err fft_err feng_qdr_err feng_chk_err adc_over noise_diode_en vacc_err rx_bad_pkt rx_bad_frame tx_over xeng_bad_dat pack_err], bitwidths=1, arith_types=2, bin_pts=0, sim_port=off, show_format=off}
      mask prompts: io_dir "I/O direction"; io_delay "I/O delay"; sample_period "Sample period"; names "Names [msb ... lsb]:"; bitwidths "Bitwidth:"; arith_types "Type (ufix=0, fix=1, bool=2):"; bin_pts "Binary pt:"; sim_port "Provide sim input/output?"; show_format "Print format string?"
      mask init:
      | swreg_init(gcb)
      settings: AttributesFormatString=14 outputs
      mask TypeOptions mode: one value | fields of equal size | fields of arbitrary size
      mask Callback mode: swreg_cb(gcb);
      mask TypeOptions io_dir: To Processor | From Processor
      mask Callback io_dir:
      | mask_enables = get_param(gcb, 'MaskEnables');
      | mask_names = get_param(gcb, 'MaskNames');
      | if strcmp(get_param(gcb, 'io_dir'), 'To Processor'),
      |     mask_enables{ismember(mask_names, 'sample_period')} = 'off';
      | else
      |     mask_enables{ismember(mask_names, 'sample_period')} = 'on';
      | end
      | set_param(gcb, 'MaskEnables', mask_enables);
      mask Callback bitwidths:
      | blk = gcb;
      | mode = get_param(blk, 'mode');
      | current_widths = eval(get_param(blk, 'bitwidths'));
      | if (strcmp(mode, 'one value') || strcmp(mode, 'fields of equal size')) && (length(current_widths) > 1),
      |     error('Only one width may be specified for this mode.');
      | elseif strcmp(mode, 'fields of arbitrary size')
      |     current_names = textscan(strtrim(strrep(strrep(get_param(blk, 'names'), ']', ''), '[', '')), '%s');
      |     current_names = current_names{1};
      |     numios = length(current_names);
      |     if length(current_widths) ~= numios,
      |         error('%d field names specified, but %d widths?', numios, length(current_widths));
      |     end
      | end
      | total_width = 0;
      | for ctr = 1 : length(current_widths),
      |     total_width = total_width + current_widths(ctr);
      | end
      | if total_width > 32,
      |     error('Total width must be 32 or less, set to %d.', total_width);
      | end
      mask Callback arith_types:
      | blk = gcb;
      | mode = get_param(blk, 'mode');
      | current_types = eval(get_param(blk, 'arith_types'));
      | numios = length(current_types);
      | if (strcmp(mode, 'one value') || strcmp(mode, 'fields of equal size')) && (length(current_types) > 1),
      |     error('Only one type may be specified for this mode.');
      | elseif strcmp(mode, 'fields of arbitrary size')
      |     current_names = textscan(strtrim(strrep(strrep(get_param(blk, 'names'), ']', ''), '[', '')), '%s');
      |     current_names = current_names{1};
      |     numios = length(current_names);
      |     if length(current_types) ~= numios,
      |         error('%d field names specified, but %d types?', numios, length(current_types));
      |     end
      | end
      | problem = 0;
      | for ctr = 1 : numios,
      |     t = current_types(ctr);
      |     if (t < 0) || (t > 2),
      |         problem = t;
      |         ctr = numios + 1;
      |     end
      | end
      | if problem ~= 0,
      |     error('Type cannot be %i, must be 0, 1 or 2.', problem);
      | end
      mask Callback bin_pts:
      | blk = gcb;
      | mode = get_param(blk, 'mode');
      | current_bins = eval(get_param(blk, 'bin_pts'));
      | if (strcmp(mode, 'one value') || strcmp(mode, 'fields of equal size')) && (length(current_bins) > 1),
      |     error('Only one binary pt may be specified for this mode.');
      | elseif strcmp(mode, 'fields of arbitrary size')
      |     current_names = textscan(strtrim(strrep(strrep(get_param(blk, 'names'), ']', ''), '[', '')), '%s');
      |     current_names = current_names{1};
      |     numios = length(current_names);
      |     if length(current_bins) ~= numios,
      |         error('%d field names specified, but %d binary pts?', numios, length(current_bins));
      |     end
      | end
  xstatus3 : Subsystem  Tag=xps:sw_reg  AncestorBlock=xps_library/software register  mask(swreg){mode=fields of equal size, io_dir=To Processor, io_delay=1, sample_period=1, names=[gbe_down rx_dest_err feng_rx_err fft_err feng_qdr_err feng_chk_err adc_over noise_diode_en vacc_err rx_bad_pkt rx_bad_frame tx_over xeng_bad_dat pack_err], bitwidths=1, arith_types=2, bin_pts=0, sim_port=off, show_format=off}
      mask prompts: io_dir "I/O direction"; io_delay "I/O delay"; sample_period "Sample period"; names "Names [msb ... lsb]:"; bitwidths "Bitwidth:"; arith_types "Type (ufix=0, fix=1, bool=2):"; bin_pts "Binary pt:"; sim_port "Provide sim input/output?"; show_format "Print format string?"
      mask init:
      | swreg_init(gcb)
      settings: AttributesFormatString=14 outputs
      mask TypeOptions mode: one value | fields of equal size | fields of arbitrary size
      mask Callback mode: swreg_cb(gcb);
      mask TypeOptions io_dir: To Processor | From Processor
      mask Callback io_dir:
      | mask_enables = get_param(gcb, 'MaskEnables');
      | mask_names = get_param(gcb, 'MaskNames');
      | if strcmp(get_param(gcb, 'io_dir'), 'To Processor'),
      |     mask_enables{ismember(mask_names, 'sample_period')} = 'off';
      | else
      |     mask_enables{ismember(mask_names, 'sample_period')} = 'on';
      | end
      | set_param(gcb, 'MaskEnables', mask_enables);
      mask Callback bitwidths:
      | blk = gcb;
      | mode = get_param(blk, 'mode');
      | current_widths = eval(get_param(blk, 'bitwidths'));
      | if (strcmp(mode, 'one value') || strcmp(mode, 'fields of equal size')) && (length(current_widths) > 1),
      |     error('Only one width may be specified for this mode.');
      | elseif strcmp(mode, 'fields of arbitrary size')
      |     current_names = textscan(strtrim(strrep(strrep(get_param(blk, 'names'), ']', ''), '[', '')), '%s');
      |     current_names = current_names{1};
      |     numios = length(current_names);
      |     if length(current_widths) ~= numios,
      |         error('%d field names specified, but %d widths?', numios, length(current_widths));
      |     end
      | end
      | total_width = 0;
      | for ctr = 1 : length(current_widths),
      |     total_width = total_width + current_widths(ctr);
      | end
      | if total_width > 32,
      |     error('Total width must be 32 or less, set to %d.', total_width);
      | end
      mask Callback arith_types:
      | blk = gcb;
      | mode = get_param(blk, 'mode');
      | current_types = eval(get_param(blk, 'arith_types'));
      | numios = length(current_types);
      | if (strcmp(mode, 'one value') || strcmp(mode, 'fields of equal size')) && (length(current_types) > 1),
      |     error('Only one type may be specified for this mode.');
      | elseif strcmp(mode, 'fields of arbitrary size')
      |     current_names = textscan(strtrim(strrep(strrep(get_param(blk, 'names'), ']', ''), '[', '')), '%s');
      |     current_names = current_names{1};
      |     numios = length(current_names);
      |     if length(current_types) ~= numios,
      |         error('%d field names specified, but %d types?', numios, length(current_types));
      |     end
      | end
      | problem = 0;
      | for ctr = 1 : numios,
      |     t = current_types(ctr);
      |     if (t < 0) || (t > 2),
      |         problem = t;
      |         ctr = numios + 1;
      |     end
      | end
      | if problem ~= 0,
      |     error('Type cannot be %i, must be 0, 1 or 2.', problem);
      | end
      mask Callback bin_pts:
      | blk = gcb;
      | mode = get_param(blk, 'mode');
      | current_bins = eval(get_param(blk, 'bin_pts'));
      | if (strcmp(mode, 'one value') || strcmp(mode, 'fields of equal size')) && (length(current_bins) > 1),
      |     error('Only one binary pt may be specified for this mode.');
      | elseif strcmp(mode, 'fields of arbitrary size')
      |     current_names = textscan(strtrim(strrep(strrep(get_param(blk, 'names'), ']', ''), '[', '')), '%s');
      |     current_names = current_names{1};
      |     numios = length(current_names);
      |     if length(current_bins) ~= numios,
      |         error('%d field names specified, but %d binary pts?', numios, length(current_bins));
      |     end
      | end
  wires:
  Subsystem5/1(rx_cnt) -> Delay66/1(d)
  [cnt_rst] -> Subsystem5/1(rst)
  miss_cnt0/2(missing_cnt) -> Convert1/1
  [cnt_rst] -> miss_cnt0/1(rst)
  Subsystem5/2(err_cnt) -> Delay67/1(d)
  miss_cnt0/1(spectr_cnt) -> Convert/1
  Delay61/1(q) -> pkt_reord_cnt0/1(out_reg)
  Delay62/1(q) -> pkt_reord_err0/1(out_reg)
  Delay66/1(q) -> rx_cnt0/1(out_reg)
  Delay67/1(q) -> rx_err_cnt0/1(out_reg)
  pkt_reord_devel0/4(time_out) -> Slice38/1, Delay26/1(d)
  pkt_reord_devel0/1(sync_out) -> Delay20/1(d), [x_sync0], snap_reord0/11(trig), miss_cnt0/2(sync), snap_reord0/1(in_sync)
  master_reset_sim4/1 -> acc_len/1(sim_1)
  acc_len/1(in_reg) -> [acc_len]
  err_clear_sim2/1 -> Subsystem2/5(data_sel)
  err_clear_sim6/1 -> Subsystem2/4(valid_sel)
  err_clear_sim7/1 -> Subsystem2/3(inj_vector)
  err_clear_sim8/1 -> Subsystem2/2(inj_counter)
  Pulse Generator1/1 -> Subsystem2/1(new_acc)
  err_clear_sim9/1 -> Subsystem2/6(run)
  Subsystem2/1(Out1) -> Terminator37/1
  Delay17/1(q) -> negedge_delay/1(in)
  xeng_tvg0/1(sync_out) -> Delay56/1(d)
  xeng_tvg0/2(data_out) -> Delay73/1(d)
  xeng_tvg0/3(valid_out) -> Delay74/1(d)
  xeng0/1(sync_out) -> snap_xeng0/3(trig), vacc_tvg0/2(sync_in)
  xeng0/2(acc) -> 16b_32b/1(In1)
  xeng0/3(valid) -> vacc_tvg0/4(valid_in), snap_xeng0/2(we)
  [xeng_tvg_sel] -> xeng_tvg0/1(tvg_sel)
  [vacc_tvg_sel] -> vacc_tvg0/1(tvg_sel)
  Delay151/1(q) -> Delay83/1(d)
  Delay20/1(q) -> xeng_tvg0/2(sync)
  Delay21/1(q) -> xeng_tvg0/3(data_in)
  Delay22/1(q) -> xeng_tvg0/4(valid_in)
  Delay26/1(q) -> Delay151/1(d)
  Delay118/1(q) -> negedge_delay1/1(in)
  16b_32b/1(Out1) -> snap_xeng0/1(din), vacc_tvg0/3(data_in)
  Delay130/1(q) -> last_missing_ant0/1(out_reg)
  miss_cnt0/3(last_missed_ant) -> Convert2/1
  [gbe_rxvld0] -> Delay6/1(d)
  [gbe_rxdata0] -> Delay2/1(d)
  [gbe_rxeof0] -> Delay7/1(d)
  Delay2/1(q) -> spead_unpack0/1(pkt_data)
  Delay6/1(q) -> spead_unpack0/2(pkt_valid)
  Delay7/1(q) -> spead_unpack0/3(pkt_eof)
  vacc_tvg0/1(sync_out) -> fake_vacc0/5(sync_in)
  vacc_tvg0/2(data_out) -> fake_vacc0/6(data_in)
  vacc_tvg0/3(valid_out) -> fake_vacc0/7(we)
  [acc_len] -> fake_vacc0/4(acc_len)
  xeng0/4(mcnt_out) -> delay5/1
  vacc_monitor/2(spec_cnt) -> vacc_cnt0/1(out_reg)
  vacc_monitor/1(error_cnt) -> vacc_err_cnt0/1(out_reg)
  fake_vacc0/1(new_acc) -> [new_acc0]
  [cnt_rst] -> vacc_monitor/1(cnt_rst)
  fake_vacc0/7(timestamp) -> delay7/1
  Delay80/1(q) -> Subsystem5/2(we)
  Delay81/1(q) -> Subsystem5/3(eof)
  Delay82/1(q) -> Subsystem5/4(flag)
  Delay56/1(q) -> xeng0/1(sync_in)
  Delay73/1(q) -> xeng0/2(ant)
  Delay74/1(q) -> xeng0/3(window_valid)
  Delay83/1(q) -> xeng0/4(mcnt_in)
  [gbe_out_rst] -> delay8/1
  [gbe_txd0] -> delay9/1
  [gbe_txvld0] -> delay10/1
  [gbe_txip] -> delay11/1
  [gbe_txport] -> delay12/1
  [gbe_txeof0] -> delay13/1
  gbe0/1(led_up) -> [gbe_up0]
  gbe0/2(led_rx) -> Terminator7/1
  gbe0/3(led_tx) -> Terminator13/1
  gbe0/4(tx_afull) -> Terminator14/1
  gbe0/5(tx_overflow) -> [gbe_tx_over0]
  gbe0/12(rx_overrun) -> Terminator36/1
  gbe0/11(rx_bad_frame) -> [gbe_rx_bad0]
  gbe0/6(rx_data) -> [gbe_rxdata0]
  gbe0/7(rx_valid) -> [gbe_rxvld0]
  gbe0/8(rx_source_ip) -> Terminator15/1
  gbe0/9(rx_source_port) -> Terminator35/1
  gbe0/10(rx_end_of_frame) -> [gbe_rxeof0]
  [vacc_ld_arm] -> fake_vacc0/2(arm)
  [vacc_ld_time] -> fake_vacc0/3(load_time)
  [vacc_rst] -> fake_vacc0/1(rst)
  delay5/1 -> fake_vacc0/8(pcnt_in)
  fake_vacc0/10(error_out) -> [vacc_err0]
  [new_acc0] -> vacc_monitor/2(new_acc)
  [vacc_err0] -> vacc_monitor/3(error)
  pkt_reord_devel0/2(data_out) -> snap_reord0/2(in_data), Delay21/1(d)
  Delay27/1(q) -> negedge_delay2/1(in)
  Delay96/1(q) -> negedge_delay3/1(in)
  Delay97/1(q) -> negedge_delay4/1(in)
  miss_cnt0/4(not_rcvd) -> [xeng_rx_err0]
  fake_vacc0/2(data_out) -> delay4/1
  fake_vacc0/4(valid_out) -> delay2/1
  fake_vacc0/6(rb_done) -> delay6/1
  [vacc_ld_stat0] -> vacc_ld_status0/1(out_reg)
  fake_vacc0/8(ld_status) -> [vacc_ld_stat0]
  [id0] -> pack_out0/6(xeng_id)
  [vacc_err0] -> snap_vacc0/4(stop)
  pack_out0/3(eof) -> Delay15/1(d)
  [cnt_rst] -> vacc_monitor2/1(cnt_rst)
  vacc_monitor2/1(pkt_cnt) -> pack_out_cnt0/1(out_reg)
  vacc_monitor2/2(error_cnt) -> pack_out_err0/1(out_reg)
  pack_out0/5(fetch) -> fake_vacc0/9(re)
  delay4/1 -> snap_vacc0/1(din), pack_out0/1(data_in)
  delay2/1 -> snap_vacc0/2(we), pack_out0/2(valid_in)
  delay6/1 -> pack_out0/4(rb_done), snap_vacc0/3(trig)
  delay7/1 -> pack_out0/5(timestamp)
  pack_out0/1(data_out) -> Delay23/1(d)
  pack_out0/2(valid_out) -> Logical/2
  pack_out0/4(err) -> Delay34/1(d)
  Delay34/1(q) -> [pack_err0], vacc_monitor2/3(error)
  delay8/1 -> gbe0/1(rst)
  delay9/1 -> gbe0/2(tx_data)
  delay10/1 -> gbe0/3(tx_valid)
  delay11/1 -> gbe0/4(tx_dest_ip)
  delay12/1 -> gbe0/5(tx_dest_port)
  delay13/1 -> gbe0/6(tx_end_of_frame)
  Constant2/1 -> gbe0/7(rx_ack)
  Constant8/1 -> gbe0/8(rx_overrun_ack)
  Delay46/1 -> pack_out0/3(pkt_rdy)
  negedge_delay3/1(out) -> front_panel/6(led2_red)
  negedge_delay4/1(out) -> front_panel/7(led3_red)
  [flasher_en] -> front_panel/1(flasher_en)
  [new_acc0] -> front_panel/2(sync)
  [x_sync0] -> front_panel/3(step)
  negedge_delay2/1(out) -> front_panel/4(led0_red)
  negedge_delay/1(out) -> front_panel/10(led6_green)
  negedge_delay1/1(out) -> front_panel/9(led5_green)
  Delay16/1 -> [gbe_txvld0]
  Delay23/1(q) -> rate_ctrl0/1(din0)
  rate_ctrl0/2(valid) -> Delay16/1
  Constant22/1 -> [beng_data_id]
  rate_ctrl0/1(dout) -> Delay114/1
  Delay114/1 -> [gbe_txd0]
  gbe_out_port/1(in_reg) -> Delay9/1(d)
  gbe_out_ip/1(in_reg) -> Delay10/1(d)
  Delay9/1(q) -> [gbe_txport]
  Delay10/1(q) -> [gbe_txip]
  [gbe_out_en] -> Logical/1
  Constant24/1 -> [beng_time_id]
  Logical/1 -> rate_ctrl0/2(valid0)
  Delay15/1(q) -> vacc_monitor2/2(eof), rate_ctrl0/3(eof0)
  fake_vacc0/5(pkt_rdy) -> rate_ctrl0/4(data_rdy0)
  spead_unpack0/1(pkt_start) -> Terminator28/1
  pre_process0/9(dest_err) -> Logical1/2, [rx_dest_err0], snap_unpack0/9(in_dest_err)
  pre_process0/1(data_out) -> pkt_reord_devel0/1(din), snap_unpack0/1(in_data)
  pre_process0/2(valid) -> snap_unpack0/15(we), pkt_reord_devel0/2(valid_in), snap_unpack0/2(in_valid)
  pre_process0/3(eof_out) -> snap_unpack0/16(trig), pkt_reord_devel0/3(eof), snap_unpack0/3(in_eof)
  pre_process0/4(timestamp) -> pkt_reord_devel0/4(time), Slice29/1
  pre_process0/5(feng_id) -> pkt_reord_devel0/5(ant), Slice30/1
  pre_process0/6(freq_out) -> Slice31/1, pkt_reord_devel0/6(freq)
  pre_process0/8(spead_err_out) -> Logical1/1, [spead_err0], snap_unpack0/8(in_spead_err)
  pre_process0/7(adc_over) -> [adc_err0], snap_unpack0/7(in_adc_over)
  pre_process0/10(fft_err) -> snap_unpack0/10(in_fft_err), [fft_err0]
  pre_process0/11(feng_rx_err) -> snap_unpack0/11(in_feng_rx_err), Logical1/3, [feng_rx_err0]
  pre_process0/12(nd_en) -> snap_unpack0/12(in_nd_en), [noise_diode_en0]
  pkt_reord_devel0/7(err) -> Terminator2/1
  pre_process0/13(chksum_err) -> snap_unpack0/13(in_chksum_err), Logical1/4, [feng_chk_err0]
  pre_process0/14(qdr_err) -> snap_unpack0/14(in_feng_qdr_err), [feng_qdr_err0]
  [id0] -> pre_process0/9(board_id)
  Constant3/1 -> Delay72/1(d)
  Delay72/1(q) -> Subsystem1/1(In1)
  Subsystem1/1(Out1) -> [id0]
  Subsystem1/2(Out2) -> [id1]
  Subsystem1/3(Out3) -> [id2]
  Subsystem1/4(Out4) -> [id3]
  [id0] -> pkt_reord_devel0/8(board_id)
  pkt_reord_devel0/3(valid_out) -> miss_cnt0/3(valid), snap_reord0/3(in_valid), snap_reord0/10(we), Logical6/2, Delay22/1(d)
  pkt_reord_devel0/5(freq_out) -> Convert12/1
  Slice12/1 -> snap_reord0/7(in_feng_err)
  Slice16/1 -> snap_reord0/9(in_nd_on)
  Slice15/1 -> snap_reord0/8(in_adc_over)
  pkt_reord_devel0/6(flag_out) -> Slice11/1, Slice12/1, Slice15/1, Slice16/1
  Slice11/1 -> miss_cnt0/4(not rcvd), snap_reord0/6(in_xeng_err), Logical6/1
  Logical6/1 -> snap_reord0/12(stop)
  miss_cnt1/2(missing_cnt) -> Convert4/1
  [cnt_rst] -> miss_cnt1/1(rst)
  miss_cnt1/1(spectr_cnt) -> Convert3/1
  pkt_reord_devel1/4(time_out) -> Slice21/1, Delay30/1(d)
  pkt_reord_devel1/1(sync_out) -> snap_reord1/11(trig), snap_reord1/1(in_sync), miss_cnt1/2(sync), Delay5/1(d)
  xeng_tvg1/1(sync_out) -> Delay32/1(d)
  xeng_tvg1/2(data_out) -> Delay36/1(d)
  xeng_tvg1/3(valid_out) -> Delay37/1(d)
  xeng1/1(sync_out) -> vacc_tvg1/2(sync_in)
  xeng1/2(acc) -> 16b_32b1/1(In1)
  xeng1/3(valid) -> vacc_tvg1/4(valid_in)
  [xeng_tvg_sel] -> xeng_tvg1/1(tvg_sel)
  [vacc_tvg_sel] -> vacc_tvg1/1(tvg_sel)
  Delay4/1(q) -> Delay38/1(d)
  Delay5/1(q) -> xeng_tvg1/2(sync)
  Delay11/1(q) -> xeng_tvg1/3(data_in)
  Delay14/1(q) -> xeng_tvg1/4(valid_in)
  Delay30/1(q) -> Delay4/1(d)
  16b_32b1/1(Out1) -> vacc_tvg1/3(data_in)
  miss_cnt1/3(last_missed_ant) -> Convert5/1
  vacc_tvg1/1(sync_out) -> fake_vacc1/5(sync_in)
  vacc_tvg1/2(data_out) -> fake_vacc1/6(data_in)
  vacc_tvg1/3(valid_out) -> fake_vacc1/7(we)
  [acc_len] -> fake_vacc1/4(acc_len)
  xeng1/4(mcnt_out) -> delay16/1
  vacc_monitor1/2(spec_cnt) -> vacc_cnt1/1(out_reg)
  vacc_monitor1/1(error_cnt) -> vacc_err_cnt1/1(out_reg)
  fake_vacc1/1(new_acc) -> vacc_monitor1/2(new_acc), [new_acc1]
  [cnt_rst] -> vacc_monitor1/1(cnt_rst)
  fake_vacc1/7(timestamp) -> delay18/1
  Delay32/1(q) -> xeng1/1(sync_in)
  Delay36/1(q) -> xeng1/2(ant)
  Delay37/1(q) -> xeng1/3(window_valid)
  Delay38/1(q) -> xeng1/4(mcnt_in)
  [vacc_ld_arm] -> fake_vacc1/2(arm)
  [vacc_ld_time] -> fake_vacc1/3(load_time)
  [vacc_rst] -> fake_vacc1/1(rst)
  delay16/1 -> fake_vacc1/8(pcnt_in)
  pkt_reord_devel1/2(data_out) -> snap_reord1/2(in_data), Delay11/1(d)
  miss_cnt1/4(not_rcvd) -> [xeng_rx_err1]
  fake_vacc1/2(data_out) -> delay3/1
  fake_vacc1/4(valid_out) -> delay1/1
  fake_vacc1/6(rb_done) -> delay17/1
  fake_vacc1/5(pkt_rdy) -> rate_ctrl1/4(data_rdy0)
  fake_vacc1/8(ld_status) -> vacc_ld_status1/1(out_reg)
  [id1] -> pack_out1/6(xeng_id)
  fake_vacc1/10(error_out) -> snap_vacc1/4(stop), vacc_monitor1/3(error), [vacc_err1]
  pack_out1/3(eof) -> Delay3/1(d)
  [cnt_rst] -> vacc_monitor3/1(cnt_rst)
  vacc_monitor3/1(pkt_cnt) -> pack_out_cnt1/1(out_reg)
  vacc_monitor3/2(error_cnt) -> pack_out_err1/1(out_reg)
  pack_out1/5(fetch) -> fake_vacc1/9(re)
  delay3/1 -> pack_out1/1(data_in), snap_vacc1/1(din)
  delay1/1 -> pack_out1/2(valid_in), snap_vacc1/2(we)
  delay17/1 -> pack_out1/4(rb_done), snap_vacc1/3(trig)
  delay18/1 -> pack_out1/5(timestamp)
  pack_out1/1(data_out) -> Delay28/1(d)
  pack_out1/2(valid_out) -> Logical7/2
  Delay28/1(q) -> rate_ctrl1/1(din0)
  Logical7/1 -> rate_ctrl1/2(valid0)
  pack_out1/4(err) -> Delay31/1(d)
  Delay3/1(q) -> vacc_monitor3/2(eof), rate_ctrl1/3(eof0)
  Delay31/1(q) -> [pack_err1], vacc_monitor3/3(error)
  Delay42/1 -> pack_out1/3(pkt_rdy)
  [gbe_out_en] -> Logical7/1
  pkt_reord_devel1/7(err) -> Terminator20/1
  [id1] -> pkt_reord_devel1/8(board_id)
  [flags1] -> pkt_reord_devel1/7(flag)
  pkt_reord_devel1/3(valid_out) -> snap_reord1/10(we), snap_reord1/3(in_valid), miss_cnt1/3(valid), Logical8/2, Delay14/1(d)
  pkt_reord_devel1/5(freq_out) -> Convert13/1
  Slice18/1 -> snap_reord1/7(in_feng_err)
  Slice20/1 -> snap_reord1/9(in_nd_on)
  Slice19/1 -> snap_reord1/8(in_adc_over)
  pkt_reord_devel1/6(flag_out) -> Slice20/1, Slice19/1, Slice18/1, Slice17/1
  Slice17/1 -> snap_reord1/6(in_xeng_err), miss_cnt1/4(not rcvd), Logical8/1
  Logical8/1 -> snap_reord1/12(stop)
  Constant6/1 -> vacc_time_lsw/1(sim_1)
  vacc_time_msw/2(in_msw) -> Concat12/1
  vacc_time_lsw/1(in_reg) -> Concat12/2
  vacc_time_msw/1(in_arm) -> [vacc_ld_arm]
  Concat12/1 -> [vacc_ld_time]
  rate_ctrl0/3(eof) -> Delay45/1
  rate_ctrl0/4(pkt_send0) -> Delay46/1
  Delay45/1 -> [gbe_txeof0]
  Delay40/1 -> [gbe_txvld1]
  rate_ctrl1/2(valid) -> Delay40/1
  rate_ctrl1/1(dout) -> Delay39/1
  Delay39/1 -> [gbe_txd1]
  rate_ctrl1/3(eof) -> Delay41/1
  rate_ctrl1/4(pkt_send0) -> Delay42/1
  Delay41/1 -> [gbe_txeof1]
  Subsystem8/1(rx_cnt) -> Delay68/1(d)
  [cnt_rst] -> Subsystem8/1(rst)
  spead_unpack0/3(valid64) -> pre_process0/2(valid_in), Delay85/1(d), pre_process1/2(valid_in), Delay80/1(d)
  spead_unpack0/6(hdr1_0x1600) -> pre_process1/5(hdr1), pre_process0/5(hdr1)
  spead_unpack0/2(data64) -> pre_process1/1(data_in), pre_process0/1(data_in)
  spead_unpack0/4(eof64) -> pre_process0/3(eof_in), Delay90/1(d), pre_process1/3(eof_in), Delay81/1(d)
  spead_unpack0/7(hdr2_0x4101) -> pre_process1/6(hdr2), pre_process0/6(hdr2)
  Subsystem8/2(err_cnt) -> Delay69/1(d)
  spead_unpack0/8(hdr3_0x4102) -> pre_process1/7(hdr3), pre_process0/7(hdr3)
  spead_unpack0/5(error) -> pre_process0/4(spead_err), Delay91/1(d), pre_process1/4(spead_err), Delay82/1(d)
  Delay85/1(q) -> Subsystem8/2(we)
  Delay90/1(q) -> Subsystem8/3(eof)
  Delay91/1(q) -> Subsystem8/4(flag)
  spead_unpack1/1(pkt_start) -> Terminator34/1
  spead_unpack0/9(hdr4_0x4103) -> pre_process1/8(hdr4), pre_process0/8(hdr4)
  pre_process1/9(dest_err) -> [rx_dest_err1]
  pre_process1/1(data_out) -> pkt_reord_devel1/1(din)
  pre_process1/2(valid) -> pkt_reord_devel1/2(valid_in)
  pre_process1/3(eof_out) -> pkt_reord_devel1/3(eof)
  pre_process1/4(timestamp) -> pkt_reord_devel1/4(time)
  pre_process1/5(feng_id) -> pkt_reord_devel1/5(ant)
  pre_process1/6(freq_out) -> pkt_reord_devel1/6(freq)
  pre_process1/8(spead_err_out) -> [spead_err1]
  pre_process1/7(adc_over) -> [adc_err1]
  pre_process1/10(fft_err) -> [fft_err1]
  pre_process1/11(feng_rx_err) -> [feng_rx_err1]
  pre_process1/12(nd_en) -> [noise_diode_en1]
  pre_process1/13(chksum_err) -> [feng_chk_err1]
  pre_process1/14(qdr_err) -> [feng_qdr_err1]
  [id1] -> pre_process1/9(board_id)
  [gbe_out_rst] -> delay21/1
  [gbe_txd1] -> delay22/1
  [gbe_txip] -> delay15/1
  [gbe_txport] -> delay19/1
  delay21/1 -> gbe1/1(rst)
  delay22/1 -> gbe1/2(tx_data)
  delay14/1 -> gbe1/3(tx_valid)
  delay15/1 -> gbe1/4(tx_dest_ip)
  delay19/1 -> gbe1/5(tx_dest_port)
  delay20/1 -> gbe1/6(tx_end_of_frame)
  Constant9/1 -> gbe1/7(rx_ack)
  Constant13/1 -> gbe1/8(rx_overrun_ack)
  gbe1/11(rx_bad_frame) -> [gbe_rx_bad1]
  gbe1/5(tx_overflow) -> [gbe_tx_over1]
  [gbe_txeof1] -> delay20/1
  [gbe_txvld1] -> delay14/1
  miss_cnt2/2(missing_cnt) -> Convert7/1
  [cnt_rst] -> miss_cnt2/1(rst)
  miss_cnt2/1(spectr_cnt) -> Convert6/1
  pkt_reord_devel3/4(time_out) -> Slice27/1, Delay111/1(d)
  pkt_reord_devel3/1(sync_out) -> Delay133/1(d), snap_reord2/11(trig), snap_reord2/1(in_sync), miss_cnt2/2(sync)
  xeng_tvg2/1(sync_out) -> Delay113/1(d)
  xeng_tvg2/2(data_out) -> Delay119/1(d)
  xeng_tvg2/3(valid_out) -> Delay120/1(d)
  xeng2/1(sync_out) -> vacc_tvg2/2(sync_in)
  xeng2/2(acc) -> 16b_32b2/1(In1)
  xeng2/3(valid) -> vacc_tvg2/4(valid_in)
  [xeng_tvg_sel] -> xeng_tvg2/1(tvg_sel)
  [vacc_tvg_sel] -> vacc_tvg2/1(tvg_sel)
  Delay124/1(q) -> Delay121/1(d)
  Delay133/1(q) -> xeng_tvg2/2(sync)
  Delay107/1(q) -> xeng_tvg2/3(data_in)
  Delay108/1(q) -> xeng_tvg2/4(valid_in)
  Delay111/1(q) -> Delay124/1(d)
  16b_32b2/1(Out1) -> vacc_tvg2/3(data_in)
  miss_cnt2/3(last_missed_ant) -> Convert8/1
  vacc_tvg2/1(sync_out) -> fake_vacc2/5(sync_in)
  vacc_tvg2/2(data_out) -> fake_vacc2/6(data_in)
  vacc_tvg2/3(valid_out) -> fake_vacc2/7(we)
  [acc_len] -> fake_vacc2/4(acc_len)
  xeng2/4(mcnt_out) -> delay26/1
  vacc_monitor4/2(spec_cnt) -> vacc_cnt2/1(out_reg)
  vacc_monitor4/1(error_cnt) -> vacc_err_cnt2/1(out_reg)
  fake_vacc2/1(new_acc) -> [new_acc2], vacc_monitor4/2(new_acc)
  [cnt_rst] -> vacc_monitor4/1(cnt_rst)
  fake_vacc2/7(timestamp) -> delay28/1
  Delay113/1(q) -> xeng2/1(sync_in)
  Delay119/1(q) -> xeng2/2(ant)
  Delay120/1(q) -> xeng2/3(window_valid)
  Delay121/1(q) -> xeng2/4(mcnt_in)
  [vacc_ld_arm] -> fake_vacc2/2(arm)
  [vacc_ld_time] -> fake_vacc2/3(load_time)
  [vacc_rst] -> fake_vacc2/1(rst)
  delay26/1 -> fake_vacc2/8(pcnt_in)
  pkt_reord_devel3/2(data_out) -> snap_reord2/2(in_data), Delay107/1(d)
  miss_cnt2/4(not_rcvd) -> [xeng_rx_err2]
  fake_vacc2/2(data_out) -> delay33/1
  fake_vacc2/4(valid_out) -> delay23/1
  fake_vacc2/6(rb_done) -> delay27/1
  fake_vacc2/5(pkt_rdy) -> rate_ctrl2/4(data_rdy0)
  fake_vacc2/8(ld_status) -> vacc_ld_status2/1(out_reg)
  [id2] -> pack_out2/6(xeng_id)
  fake_vacc2/10(error_out) -> [vacc_err2], vacc_monitor4/3(error), snap_vacc2/4(stop)
  pack_out2/3(eof) -> Delay110/1(d)
  [cnt_rst] -> vacc_monitor5/1(cnt_rst)
  vacc_monitor5/1(pkt_cnt) -> pack_out_cnt2/1(out_reg)
  vacc_monitor5/2(error_cnt) -> pack_out_err2/1(out_reg)
  pack_out2/5(fetch) -> fake_vacc2/9(re)
  delay33/1 -> snap_vacc2/1(din), pack_out2/1(data_in)
  delay23/1 -> snap_vacc2/2(we), pack_out2/2(valid_in)
  delay27/1 -> snap_vacc2/3(trig), pack_out2/4(rb_done)
  delay28/1 -> pack_out2/5(timestamp)
  pack_out2/1(data_out) -> Delay109/1(d)
  pack_out2/2(valid_out) -> Logical12/2
  Delay109/1(q) -> rate_ctrl2/1(din0)
  Logical12/1 -> rate_ctrl2/2(valid0)
  pack_out2/4(err) -> Delay112/1(d)
  Delay110/1(q) -> rate_ctrl2/3(eof0), vacc_monitor5/2(eof)
  Delay112/1(q) -> [pack_err2], vacc_monitor5/3(error)
  Delay127/1 -> pack_out2/3(pkt_rdy)
  [gbe_out_en] -> Logical12/1
  pkt_reord_devel3/7(err) -> Terminator40/1
  [id2] -> pkt_reord_devel3/8(board_id)
  [flags2] -> pkt_reord_devel3/7(flag)
  pkt_reord_devel3/3(valid_out) -> Delay108/1(d), Logical13/2, snap_reord2/10(we), miss_cnt2/3(valid), snap_reord2/3(in_valid)
  pkt_reord_devel3/5(freq_out) -> Convert14/1
  Slice24/1 -> snap_reord2/7(in_feng_err)
  Slice26/1 -> snap_reord2/9(in_nd_on)
  Slice25/1 -> snap_reord2/8(in_adc_over)
  pkt_reord_devel3/6(flag_out) -> Slice26/1, Slice25/1, Slice23/1, Slice24/1
  Slice23/1 -> Logical13/1, snap_reord2/6(in_xeng_err), miss_cnt2/4(not rcvd)
  Logical13/1 -> snap_reord2/12(stop)
  Delay125/1 -> [gbe_txvld2]
  rate_ctrl2/2(valid) -> Delay125/1
  rate_ctrl2/1(dout) -> Delay123/1
  Delay123/1 -> [gbe_txd2]
  rate_ctrl2/3(eof) -> Delay126/1
  rate_ctrl2/4(pkt_send0) -> Delay127/1
  Delay126/1 -> [gbe_txeof2]
  Subsystem11/1(rx_cnt) -> Delay149/1(d)
  [cnt_rst] -> Subsystem11/1(rst)
  Subsystem11/2(err_cnt) -> Delay150/1(d)
  Delay149/1(q) -> rx_cnt2/1(out_reg)
  Delay150/1(q) -> rx_err_cnt2/1(out_reg)
  Delay155/1(q) -> Subsystem11/2(we)
  Delay156/1(q) -> Subsystem11/3(eof)
  Delay157/1(q) -> Subsystem11/4(flag)
  pre_process2/9(dest_err) -> [rx_dest_err2]
  pre_process2/1(data_out) -> pkt_reord_devel3/1(din)
  pre_process2/2(valid) -> pkt_reord_devel3/2(valid_in)
  pre_process2/3(eof_out) -> pkt_reord_devel3/3(eof)
  pre_process2/4(timestamp) -> pkt_reord_devel3/4(time)
  pre_process2/5(feng_id) -> pkt_reord_devel3/5(ant)
  pre_process2/6(freq_out) -> pkt_reord_devel3/6(freq)
  pre_process2/8(spead_err_out) -> [spead_err2]
  pre_process2/7(adc_over) -> [adc_err2]
  pre_process2/10(fft_err) -> [fft_err2]
  pre_process2/11(feng_rx_err) -> [feng_rx_err2]
  pre_process2/12(nd_en) -> [noise_diode_en2]
  pre_process2/13(chksum_err) -> [feng_chk_err2]
  pre_process2/14(qdr_err) -> [feng_qdr_err2]
  [id2] -> pre_process2/9(board_id)
  miss_cnt3/2(missing_cnt) -> Convert10/1
  [cnt_rst] -> miss_cnt3/1(rst)
  miss_cnt3/1(spectr_cnt) -> Convert9/1
  pkt_reord_devel4/4(time_out) -> Slice36/1, Delay171/1(d)
  pkt_reord_devel4/1(sync_out) -> Delay188/1(d), snap_reord3/11(trig), snap_reord3/1(in_sync), miss_cnt3/2(sync)
  xeng_tvg3/1(sync_out) -> Delay173/1(d)
  xeng_tvg3/2(data_out) -> Delay176/1(d)
  xeng_tvg3/3(valid_out) -> Delay177/1(d)
  xeng3/1(sync_out) -> vacc_tvg3/2(sync_in)
  xeng3/2(acc) -> 16b_32b3/1(In1)
  xeng3/3(valid) -> vacc_tvg3/4(valid_in)
  [xeng_tvg_sel] -> xeng_tvg3/1(tvg_sel)
  [vacc_tvg_sel] -> vacc_tvg3/1(tvg_sel)
  Delay180/1(q) -> Delay178/1(d)
  Delay188/1(q) -> xeng_tvg3/2(sync)
  Delay167/1(q) -> xeng_tvg3/3(data_in)
  Delay168/1(q) -> xeng_tvg3/4(valid_in)
  Delay171/1(q) -> Delay180/1(d)
  16b_32b3/1(Out1) -> vacc_tvg3/3(data_in)
  miss_cnt3/3(last_missed_ant) -> Convert11/1
  vacc_tvg3/1(sync_out) -> fake_vacc3/5(sync_in)
  vacc_tvg3/2(data_out) -> fake_vacc3/6(data_in)
  vacc_tvg3/3(valid_out) -> fake_vacc3/7(we)
  [acc_len] -> fake_vacc3/4(acc_len)
  xeng3/4(mcnt_out) -> delay37/1
  vacc_monitor6/2(spec_cnt) -> vacc_cnt3/1(out_reg)
  vacc_monitor6/1(error_cnt) -> vacc_err_cnt3/1(out_reg)
  fake_vacc3/1(new_acc) -> vacc_monitor6/2(new_acc), [new_acc3]
  [cnt_rst] -> vacc_monitor6/1(cnt_rst)
  fake_vacc3/7(timestamp) -> delay39/1
  Delay173/1(q) -> xeng3/1(sync_in)
  Delay176/1(q) -> xeng3/2(ant)
  Delay177/1(q) -> xeng3/3(window_valid)
  Delay178/1(q) -> xeng3/4(mcnt_in)
  [vacc_ld_arm] -> fake_vacc3/2(arm)
  [vacc_ld_time] -> fake_vacc3/3(load_time)
  [vacc_rst] -> fake_vacc3/1(rst)
  delay37/1 -> fake_vacc3/8(pcnt_in)
  pkt_reord_devel4/2(data_out) -> snap_reord3/2(in_data), Delay167/1(d)
  miss_cnt3/4(not_rcvd) -> [xeng_rx_err3]
  fake_vacc3/2(data_out) -> delay44/1
  fake_vacc3/4(valid_out) -> delay34/1
  fake_vacc3/6(rb_done) -> delay38/1
  fake_vacc3/5(pkt_rdy) -> rate_ctrl3/4(data_rdy0)
  fake_vacc3/8(ld_status) -> vacc_ld_status3/1(out_reg)
  [id3] -> pack_out3/6(xeng_id)
  fake_vacc3/10(error_out) -> snap_vacc3/4(stop), vacc_monitor6/3(error), [vacc_err3]
  pack_out3/3(eof) -> Delay170/1(d)
  [cnt_rst] -> vacc_monitor7/1(cnt_rst)
  vacc_monitor7/1(pkt_cnt) -> pack_out_cnt3/1(out_reg)
  vacc_monitor7/2(error_cnt) -> pack_out_err3/1(out_reg)
  pack_out3/5(fetch) -> fake_vacc3/9(re)
  delay44/1 -> pack_out3/1(data_in), snap_vacc3/1(din)
  delay34/1 -> pack_out3/2(valid_in), snap_vacc3/2(we)
  delay38/1 -> pack_out3/4(rb_done), snap_vacc3/3(trig)
  delay39/1 -> pack_out3/5(timestamp)
  pack_out3/1(data_out) -> Delay169/1(d)
  pack_out3/2(valid_out) -> Logical16/2
  Delay169/1(q) -> rate_ctrl3/1(din0)
  Logical16/1 -> rate_ctrl3/2(valid0)
  pack_out3/4(err) -> Delay172/1(d)
  Delay170/1(q) -> vacc_monitor7/2(eof), rate_ctrl3/3(eof0)
  Delay172/1(q) -> [pack_err3], vacc_monitor7/3(error)
  Delay183/1 -> pack_out3/3(pkt_rdy)
  [gbe_out_en] -> Logical16/1
  pkt_reord_devel4/7(err) -> Terminator57/1
  [id3] -> pkt_reord_devel4/8(board_id)
  [flags3] -> pkt_reord_devel4/7(flag)
  pkt_reord_devel4/3(valid_out) -> snap_reord3/10(we), snap_reord3/3(in_valid), miss_cnt3/3(valid), Logical17/2, Delay168/1(d)
  pkt_reord_devel4/5(freq_out) -> Convert15/1
  Slice33/1 -> snap_reord3/7(in_feng_err)
  Slice35/1 -> snap_reord3/9(in_nd_on)
  Slice34/1 -> snap_reord3/8(in_adc_over)
  pkt_reord_devel4/6(flag_out) -> Slice35/1, Slice34/1, Slice33/1, Slice32/1
  Slice32/1 -> snap_reord3/6(in_xeng_err), miss_cnt3/4(not rcvd), Logical17/1
  Logical17/1 -> snap_reord3/12(stop)
  Delay181/1 -> [gbe_txvld3]
  rate_ctrl3/2(valid) -> Delay181/1
  rate_ctrl3/1(dout) -> Delay179/1
  Delay179/1 -> [gbe_txd3]
  rate_ctrl3/3(eof) -> Delay182/1
  rate_ctrl3/4(pkt_send0) -> Delay183/1
  Delay182/1 -> [gbe_txeof3]
  Subsystem14/1(rx_cnt) -> Delay195/1(d)
  [cnt_rst] -> Subsystem14/1(rst)
  spead_unpack1/3(valid64) -> Delay200/1(d), pre_process3/2(valid_in), Delay155/1(d), pre_process2/2(valid_in)
  spead_unpack1/6(hdr1_0x1600) -> pre_process3/5(hdr1), pre_process2/5(hdr1)
  spead_unpack1/2(data64) -> pre_process3/1(data_in), pre_process2/1(data_in)
  spead_unpack1/4(eof64) -> Delay201/1(d), pre_process3/3(eof_in), Delay156/1(d), pre_process2/3(eof_in)
  spead_unpack1/7(hdr2_0x4101) -> pre_process3/6(hdr2), pre_process2/6(hdr2)
  Subsystem14/2(err_cnt) -> Delay196/1(d)
  Delay195/1(q) -> rx_cnt3/1(out_reg)
  Delay196/1(q) -> rx_err_cnt3/1(out_reg)
  spead_unpack1/8(hdr3_0x4102) -> pre_process3/7(hdr3), pre_process2/7(hdr3)
  spead_unpack1/5(error) -> Delay202/1(d), pre_process3/4(spead_err), Delay157/1(d), pre_process2/4(spead_err)
  Delay200/1(q) -> Subsystem14/2(we)
  Delay201/1(q) -> Subsystem14/3(eof)
  Delay202/1(q) -> Subsystem14/4(flag)
  spead_unpack1/9(hdr4_0x4103) -> pre_process3/8(hdr4), pre_process2/8(hdr4)
  pre_process3/9(dest_err) -> [rx_dest_err3]
  pre_process3/1(data_out) -> pkt_reord_devel4/1(din)
  pre_process3/2(valid) -> pkt_reord_devel4/2(valid_in)
  pre_process3/3(eof_out) -> pkt_reord_devel4/3(eof)
  pre_process3/4(timestamp) -> pkt_reord_devel4/4(time)
  pre_process3/5(feng_id) -> pkt_reord_devel4/5(ant)
  pre_process3/6(freq_out) -> pkt_reord_devel4/6(freq)
  pre_process3/8(spead_err_out) -> [spead_err3]
  pre_process3/7(adc_over) -> [adc_err3]
  pre_process3/11(feng_rx_err) -> [feng_rx_err3]
  pre_process3/12(nd_en) -> [noise_diode_en3]
  pre_process3/13(chksum_err) -> [feng_chk_err3]
  pre_process3/14(qdr_err) -> [feng_qdr_err3]
  [id3] -> pre_process3/9(board_id)
  gbe1/1(led_up) -> [gbe_up1]
  [flags0] -> pkt_reord_devel0/7(flag)
  Delay209/1(q) -> negedge_delay5/1(in)
  Delay210/1(q) -> negedge_delay6/1(in)
  negedge_delay6/1(out) -> front_panel/8(led4_green)
  negedge_delay5/1(out) -> front_panel/5(led1_red)
  Delay211/1(q) -> negedge_delay7/1(in)
  negedge_delay7/1(out) -> front_panel/11(led7_green)
  [err0] -> Delay27/1(d)
  [data_in_bad0] -> Inverter3/1
  [data_in_bad1] -> Inverter4/1
  [data_in_bad2] -> Inverter7/1
  [data_in_bad3] -> Inverter8/1
  Inverter3/1 -> Delay210/1(d)
  Inverter4/1 -> Delay118/1(d)
  Inverter7/1 -> Delay17/1(d)
  Inverter8/1 -> Delay211/1(d)
  [err1] -> Delay209/1(d)
  [err2] -> Delay96/1(d)
  [err3] -> Delay97/1(d)
  pre_process3/10(fft_err) -> [fft_err3]
  Delay68/1(q) -> rx_cnt1/1(out_reg)
  Delay69/1(q) -> rx_err_cnt1/1(out_reg)
  Slice21/1 -> snap_reord1/4(in_time)
  Convert13/1 -> snap_reord1/5(in_freq)
  Slice27/1 -> snap_reord2/4(in_time)
  Convert14/1 -> snap_reord2/5(in_freq)
  Slice36/1 -> snap_reord3/4(in_time)
  Convert15/1 -> snap_reord3/5(in_freq)
  Slice38/1 -> snap_reord0/4(in_time)
  Convert12/1 -> snap_reord0/5(in_freq)
  Convert/1 -> Delay61/1(d)
  Convert1/1 -> Delay62/1(d)
  Convert2/1 -> Delay130/1(d)
  Delay24/1(q) -> pkt_reord_cnt1/1(out_reg)
  Delay33/1(q) -> pkt_reord_err1/1(out_reg)
  Delay1/1(q) -> last_missing_ant1/1(out_reg)
  Convert3/1 -> Delay24/1(d)
  Convert4/1 -> Delay33/1(d)
  Convert5/1 -> Delay1/1(d)
  Delay43/1(q) -> pkt_reord_cnt2/1(out_reg)
  Delay47/1(q) -> pkt_reord_err2/1(out_reg)
  Delay35/1(q) -> last_missing_ant2/1(out_reg)
  Convert6/1 -> Delay43/1(d)
  Convert7/1 -> Delay47/1(d)
  Convert8/1 -> Delay35/1(d)
  Delay49/1(q) -> pkt_reord_cnt3/1(out_reg)
  Delay50/1(q) -> pkt_reord_err3/1(out_reg)
  Delay48/1(q) -> last_missing_ant3/1(out_reg)
  Convert9/1 -> Delay49/1(d)
  Convert10/1 -> Delay50/1(d)
  Convert11/1 -> Delay48/1(d)
  Slice29/1 -> snap_unpack0/4(in_time)
  Slice30/1 -> snap_unpack0/5(in_feng_id)
  Slice31/1 -> snap_unpack0/6(in_freq)
  Logical1/1 -> snap_unpack0/17(stop)
  ctrl/3(in_cnt_rst) -> edge_detect/1(in)
  ctrl/1(in_vacc_rst) -> pipeline/1(d)
  ctrl/2(in_clr_status) -> pipeline1/1(d)
  ctrl/4(in_gbe_en) -> pipeline3/1(d)
  ctrl/5(in_gbe_rst) -> pipeline4/1(d)
  ctrl/6(in_gbe_out_en) -> pipeline5/1(d)
  ctrl/7(in_gbe_out_rst) -> pipeline6/1(d)
  ctrl/8(in_loopback_rst) -> pipeline7/1(d)
  ctrl/9(in_flasher_en) -> pipeline8/1(d)
  edge_detect/1(out) -> pipeline2/1(d)
  pipeline8/1(q) -> [flasher_en]
  pipeline7/1(q) -> [loopback_mux_rst]
  pipeline6/1(q) -> [gbe_out_rst]
  pipeline5/1(q) -> [gbe_out_en]
  pipeline4/1(q) -> [gbe_rst]
  pipeline3/1(q) -> [gbe_en]
  pipeline2/1(q) -> [cnt_rst]
  pipeline1/1(q) -> [clr_status]
  pipeline/1(q) -> [vacc_rst]
  tvg_sel/1(in_xaui) -> pipeline9/1(d)
  tvg_sel/2(in_descr) -> pipeline10/1(d)
  tvg_sel/3(in_xeng) -> pipeline12/1(d)
  tvg_sel/4(in_vacc) -> pipeline11/1(d)
  pipeline9/1(q) -> [xaui_tvg_sel]
  pipeline10/1(q) -> [descr_tvg_sel]
  pipeline12/1(q) -> [xeng_tvg_sel]
  pipeline11/1(q) -> [vacc_tvg_sel]
  pipeline13/1(q) -> [gbe_debug_rst]
  ctrl/10(in_gbe_debug_rst) -> pipeline13/1(d)
  [gbe_debug_rst] -> gbe0/9(debug_rst)
  [gbe_debug_rst] -> gbe1/9(debug_rst)
  gbe1/2(led_rx) -> Terminator38/1
  gbe1/3(led_tx) -> Terminator50/1
  gbe1/4(tx_afull) -> Terminator51/1
  gbe1/8(rx_source_ip) -> Terminator52/1
  gbe1/9(rx_source_port) -> Terminator53/1
  gbe1/12(rx_overrun) -> Terminator54/1
  [gbe_rxvld1] -> Delay12/1(d)
  [gbe_rxdata1] -> Delay8/1(d)
  [gbe_rxeof1] -> Delay13/1(d)
  Delay12/1(q) -> spead_unpack1/2(pkt_valid)
  Delay13/1(q) -> spead_unpack1/3(pkt_eof)
  Delay8/1(q) -> spead_unpack1/1(pkt_data)
  gbe1/6(rx_data) -> [gbe_rxdata1]
  gbe1/7(rx_valid) -> [gbe_rxvld1]
  gbe1/10(rx_end_of_frame) -> [gbe_rxeof1]
  [gbe_up0] -> Inverter9/1
  [clr_status] -> latch0/1(reset)
  [pack_err0] -> latch0/15(pack_err)
  latch0/12(Out12) -> xstatus0/12(out_tx_over)
  latch0/14(Out14) -> xstatus0/14(out_pack_err)
  latch0/10(Out10) -> xstatus0/10(out_rx_bad_pkt)
  latch0/11(Out11) -> xstatus0/11(out_rx_bad_frame)
  latch0/9(Out9) -> xstatus0/9(out_vacc_err)
  latch0/13(Out13) -> xstatus0/13(out_xeng_bad_dat)
  latch0/4(Out4) -> xstatus0/4(out_fft_err)
  latch0/6(Out6) -> xstatus0/6(out_feng_chk_err)
  latch0/8(Out8) -> xstatus0/8(out_noise_diode_en)
  latch0/7(Out7) -> xstatus0/7(out_adc_over)
  latch0/3(Out3) -> xstatus0/3(out_feng_rx_err)
  latch0/2(Out2) -> xstatus0/2(out_rx_dest_err)
  latch0/5(Out5) -> xstatus0/5(out_feng_qdr_err)
  latch0/1(Out1) -> xstatus0/1(out_gbe_down)
  latch0/15(data_bad) -> [data_in_bad0]
  latch0/16(error) -> [err0]
  latch0/17(flags) -> [flags0]
  Inverter9/1 -> latch0/2(gbe_down)
  [rx_dest_err0] -> latch0/3(rx_dest_err)
  [feng_rx_err0] -> latch0/4(feng_rx_err)
  [noise_diode_en0] -> latch0/9(noise_diode_en)
  [adc_err0] -> latch0/8(adc_over)
  [vacc_err0] -> latch0/10(vacc_err)
  [spead_err0] -> latch0/11(rx_bad_pkt)
  [feng_chk_err0] -> latch0/7(feng_chk_err)
  [gbe_rx_bad0] -> latch0/12(rx_bad_frame)
  [feng_qdr_err0] -> latch0/6(feng_qdr_err)
  [gbe_tx_over0] -> latch0/13(tx_over)
  [fft_err0] -> latch0/5(fft_err)
  [xeng_rx_err0] -> latch0/14(xeng_bad_dat)
  [gbe_up0] -> Inverter5/1
  [clr_status] -> latch1/1(reset)
  [pack_err1] -> latch1/15(pack_err)
  latch1/12(Out12) -> xstatus1/12(out_tx_over)
  latch1/14(Out14) -> xstatus1/14(out_pack_err)
  latch1/10(Out10) -> xstatus1/10(out_rx_bad_pkt)
  latch1/11(Out11) -> xstatus1/11(out_rx_bad_frame)
  latch1/9(Out9) -> xstatus1/9(out_vacc_err)
  latch1/13(Out13) -> xstatus1/13(out_xeng_bad_dat)
  latch1/4(Out4) -> xstatus1/4(out_fft_err)
  latch1/6(Out6) -> xstatus1/6(out_feng_chk_err)
  latch1/8(Out8) -> xstatus1/8(out_noise_diode_en)
  latch1/7(Out7) -> xstatus1/7(out_adc_over)
  latch1/3(Out3) -> xstatus1/3(out_feng_rx_err)
  latch1/2(Out2) -> xstatus1/2(out_rx_dest_err)
  latch1/5(Out5) -> xstatus1/5(out_feng_qdr_err)
  latch1/1(Out1) -> xstatus1/1(out_gbe_down)
  latch1/15(data_bad) -> [data_in_bad1]
  latch1/16(error) -> [err1]
  latch1/17(flags) -> [flags1]
  Inverter5/1 -> latch1/2(gbe_down)
  [rx_dest_err1] -> latch1/3(rx_dest_err)
  [feng_rx_err1] -> latch1/4(feng_rx_err)
  [noise_diode_en1] -> latch1/9(noise_diode_en)
  [adc_err1] -> latch1/8(adc_over)
  [vacc_err1] -> latch1/10(vacc_err)
  [spead_err1] -> latch1/11(rx_bad_pkt)
  [feng_chk_err1] -> latch1/7(feng_chk_err)
  [gbe_rx_bad0] -> latch1/12(rx_bad_frame)
  [feng_qdr_err1] -> latch1/6(feng_qdr_err)
  [gbe_tx_over0] -> latch1/13(tx_over)
  [fft_err1] -> latch1/5(fft_err)
  [xeng_rx_err1] -> latch1/14(xeng_bad_dat)
  [gbe_up1] -> Inverter1/1
  [clr_status] -> latch2/1(reset)
  [pack_err2] -> latch2/15(pack_err)
  latch2/12(Out12) -> xstatus2/12(out_tx_over)
  latch2/14(Out14) -> xstatus2/14(out_pack_err)
  latch2/10(Out10) -> xstatus2/10(out_rx_bad_pkt)
  latch2/11(Out11) -> xstatus2/11(out_rx_bad_frame)
  latch2/9(Out9) -> xstatus2/9(out_vacc_err)
  latch2/13(Out13) -> xstatus2/13(out_xeng_bad_dat)
  latch2/4(Out4) -> xstatus2/4(out_fft_err)
  latch2/6(Out6) -> xstatus2/6(out_feng_chk_err)
  latch2/8(Out8) -> xstatus2/8(out_noise_diode_en)
  latch2/7(Out7) -> xstatus2/7(out_adc_over)
  latch2/3(Out3) -> xstatus2/3(out_feng_rx_err)
  latch2/2(Out2) -> xstatus2/2(out_rx_dest_err)
  latch2/5(Out5) -> xstatus2/5(out_feng_qdr_err)
  latch2/1(Out1) -> xstatus2/1(out_gbe_down)
  latch2/15(data_bad) -> [data_in_bad2]
  latch2/16(error) -> [err2]
  latch2/17(flags) -> [flags2]
  Inverter1/1 -> latch2/2(gbe_down)
  [rx_dest_err2] -> latch2/3(rx_dest_err)
  [feng_rx_err2] -> latch2/4(feng_rx_err)
  [noise_diode_en2] -> latch2/9(noise_diode_en)
  [adc_err2] -> latch2/8(adc_over)
  [vacc_err2] -> latch2/10(vacc_err)
  [spead_err2] -> latch2/11(rx_bad_pkt)
  [feng_chk_err2] -> latch2/7(feng_chk_err)
  [gbe_rx_bad1] -> latch2/12(rx_bad_frame)
  [feng_qdr_err2] -> latch2/6(feng_qdr_err)
  [gbe_tx_over1] -> latch2/13(tx_over)
  [fft_err2] -> latch2/5(fft_err)
  [xeng_rx_err2] -> latch2/14(xeng_bad_dat)
  [gbe_up1] -> Inverter2/1
  [clr_status] -> latch3/1(reset)
  [pack_err3] -> latch3/15(pack_err)
  latch3/12(Out12) -> xstatus3/12(out_tx_over)
  latch3/14(Out14) -> xstatus3/14(out_pack_err)
  latch3/10(Out10) -> xstatus3/10(out_rx_bad_pkt)
  latch3/11(Out11) -> xstatus3/11(out_rx_bad_frame)
  latch3/9(Out9) -> xstatus3/9(out_vacc_err)
  latch3/13(Out13) -> xstatus3/13(out_xeng_bad_dat)
  latch3/4(Out4) -> xstatus3/4(out_fft_err)
  latch3/6(Out6) -> xstatus3/6(out_feng_chk_err)
  latch3/8(Out8) -> xstatus3/8(out_noise_diode_en)
  latch3/7(Out7) -> xstatus3/7(out_adc_over)
  latch3/3(Out3) -> xstatus3/3(out_feng_rx_err)
  latch3/2(Out2) -> xstatus3/2(out_rx_dest_err)
  latch3/5(Out5) -> xstatus3/5(out_feng_qdr_err)
  latch3/1(Out1) -> xstatus3/1(out_gbe_down)
  latch3/15(data_bad) -> [data_in_bad3]
  latch3/16(error) -> [err3]
  latch3/17(flags) -> [flags3]
  Inverter2/1 -> latch3/2(gbe_down)
  [rx_dest_err3] -> latch3/3(rx_dest_err)
  [feng_rx_err3] -> latch3/4(feng_rx_err)
  [noise_diode_en3] -> latch3/9(noise_diode_en)
  [adc_err3] -> latch3/8(adc_over)
  [vacc_err3] -> latch3/10(vacc_err)
  [spead_err3] -> latch3/11(rx_bad_pkt)
  [feng_chk_err3] -> latch3/7(feng_chk_err)
  [gbe_rx_bad1] -> latch3/12(rx_bad_frame)
  [feng_qdr_err3] -> latch3/6(feng_qdr_err)
  [gbe_tx_over1] -> latch3/13(tx_over)
  [fft_err3] -> latch3/5(fft_err)
  [xeng_rx_err3] -> latch3/14(xeng_bad_dat)
